simulink model "ENV"  (R2024b)
settings: Solver=FixedStepDiscrete  StartTime=0.0  StopTime=1  FixedStep=0.001  RelTol=1e-3  EnableMultiTasking=on
libraries: stm32blockslib x92, canmsglib x40, simulink x7, stm32f4xxblockslib x6
(part 1 of 5)
settings Model: DataDictionary=Master_Dictionary.sldd  STM32="{\"DigitalPortRead\":[{\"ID\":\"ENV:620\"},{\"ID\":\"ENV:1851\"},{\"ID\":\"ENV:1904\"},{\"ID\":\"ENV:2058\"}],\"SPIControllerTransfer\":[{\"ID\":\"ENV:1674\"},{\"ID\":\"ENV:1677\"},{\"ID\":\"ENV:1680\"},{\"ID\":\"ENV:1683\"},{\"ID\":\"ENV:1686\"},{\"ID\":\"ENV:1689\"},{\"ID\":\"ENV:1787\"},{\"ID\":\"ENV:1788\"},{\"ID\":\"ENV:1789\"},{\"ID\":\"ENV:1790\"},{\"ID\":\"ENV:1791\"},{\"ID\":\"ENV:1792\"},{\"ID\":\"ENV:1879\"},{\"ID\":\"ENV:1925\"},{\"ID\":\"ENV:1937\"},{\"ID\":\"ENV:1944\"},{\"ID\":\"ENV:1958\"},{\"ID\":\"ENV:1959\"},{\"ID\":\"ENV:1960\"},{\"ID\":\"ENV:1961\"},{\"ID\":\"ENV:2022\"},{\"ID\":\"ENV:2023\"},{\"ID\":\"ENV:2024\"},{\"ID\":\"ENV:2025\"},{\"ID\":\"ENV:2026\"},{\"ID\":\"ENV:2027\"},{\"ID\":\"ENV:2028\"},{\"ID\":\"ENV:2029\"},{\"ID\":\"ENV:2111\"},{\"ID\":\"ENV:2112\"},{\"ID\":\"ENV:2113\"},{\"ID\":\"ENV:2114\"},{\"ID\":\"ENV:2244\"},{\"ID\":\"ENV:2245\"},{\"ID\":\"ENV:2246\"},{\"ID\":\"ENV:2247\"},{\"ID\":\"ENV:2283\"},{\"ID\":\"ENV:2284\"},{\"ID\":\"ENV:2317\"},{\"ID\":\"ENV:2318\"},{\"ID\":\"ENV:2351\"},{\"ID\":\"ENV:2352\"},{\"ID\":\"ENV:2373\"},{\"ID\":\"ENV:2374\"},{\"ID\":\"ENV:2375\"},{\"ID\":\"ENV:2376\"},{\"ID\":\"ENV:2377\"},{\"ID\":\"ENV:2378\"},{\"ID\":\"ENV:2379\"},{\"ID\":\"ENV:2380\"},{\"ID\":\"ENV:2381\"},{\"ID\":\"ENV:2382\"},{\"ID\":\"ENV:2383\"},{\"ID\":\"ENV:2384\"},{\"ID\":\"ENV:2385\"},{\"ID\":\"ENV:2386\"},{\"ID\":\"ENV:2387\"},{\"ID\":\"ENV:2388\"},{\"ID\":\"ENV:2389\"},{\"ID\":\"ENV:2390\"},{\"ID\":\"ENV:2412\"},{\"ID\":\"ENV:2413\"},{\"ID\":\"ENV:2414\"},{\"ID\":\"ENV:2415\"},{\"ID\":\"ENV:2416\"},{\"ID\":\"ENV:2417\"},{\"ID\":\"ENV:2418\"},{\"ID\":\"ENV:2419\"},{\"ID\":\"ENV:3078\"},{\"ID\":\"ENV:3079\"},{\"ID\":\"ENV:3080\"},{\"ID\":\"ENV:3081\"},{\"ID\":\"ENV:3082\"},{\"ID\":\"ENV:3083\"},{\"ID\":\"ENV:3084\"},{\"ID\":\"ENV:3085\"},{\"ID\":\"ENV:3157\"},{\"ID\":\"ENV:3158\"},{\"ID\":\"ENV:3159\"},{\"ID\":\"ENV:3160\"},{\"ID\":\"ENV:3161\"},{\"ID\":\"ENV:3162\"},{\"ID\":\"ENV:3163\"},{\"ID\":\"ENV:3164\"},{\"ID\":\"ENV:3234\"},{\"ID\":\"ENV:3235\"},{\"ID\":\"ENV:3236\"},{\"ID\":\"ENV:3237\"},{\"ID\":\"ENV:3238\"},{\"ID\":\"ENV:3239\"},{\"ID\":\"ENV:3240\"},{\"ID\":\"ENV:3241\"}],\"DigitalPortWrite\":[{\"ID\":\"ENV:889\"},{\"ID\":\"ENV:2393\"}]}"  Creator=will  LastModifiedBy=Will
settings SolverCC: AlgebraicLoopSolver=TrustRegion
settings DataIOCC: ReturnWorkspaceOutputs=off
settings OptimizationCC: DefaultParameterBehavior=Inlined  EnhancedBackFolding=on  PassReuseOutputArgsAs=Individual arguments  ZeroExternalMemoryAtStartup=off  ZeroInternalMemoryAtStartup=off  MaxStackSize=512  OptimizeBlockOrder=speed  DifferentSizesBufferReuse=on  OptimizationCustomize=off  EfficientTunableParamExpr=on
settings DebuggingCC: ParameterTunabilityLossMsg=error  UnconnectedInputMsg=warning  UnconnectedOutputMsg=warning  UnconnectedLineMsg=warning  ArithmeticOperatorsInVariantConditions=warning
settings HardwareCC: ProdBitPerPointer=32  ProdBitPerSizeT=32  ProdBitPerPtrDiffT=32  ProdLargestAtomicInteger=Long  ProdLargestAtomicFloat=Double  ProdWordSize=32  ProdLongLongMode=on  ProdHWDeviceType=ARM Compatible->ARM Cortex-M
settings ModelReferenceCC: EnableRefExpFcnMdlSchedulingChecks=on
settings SFSimCC: MATLABDynamicMemAlloc=off  CustomCodeUndefinedFunction=UseInterfaceOnly
settings RTWCC: Description=Embedded Coder  SystemTargetFile=ert.tlc  HardwareBoard=STM32H7xx Based (Single-core)  TemplateMakefile=ert_default_tmf  CustomHeaderCode="#include \"stm32h7xx_ll_tim.h\""  CustomInitializer=LL_TIM_EnableCounter(TIM2);  Toolchain=GNU Tools for ARM Embedded Processors  GPUComputeCapability=3.5
settings CodeAppCC: ForceParamTrailComments=on  IgnoreCustomStorageClasses=off  OperatorAnnotations=on  SimulinkDataObjDesc=on  SFDataObjDesc=on  InsertBlockDesc=on
settings ERTTargetCC: TargetLangStandard=C99 (ISO)  CodeReplacementLibrary=ARM Cortex-M  ExtModeTransport=3  ExtModeStaticAlloc=on  ExtModeStaticAllocSize=2048  ExtModeMexFile=ext_xcp  ExtModeIntrfLevel=Level2 - Open

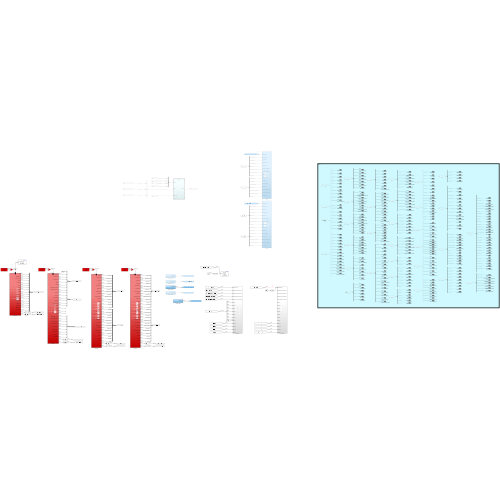
[thumbnail: Simulink's stored preview of the top-level diagram]
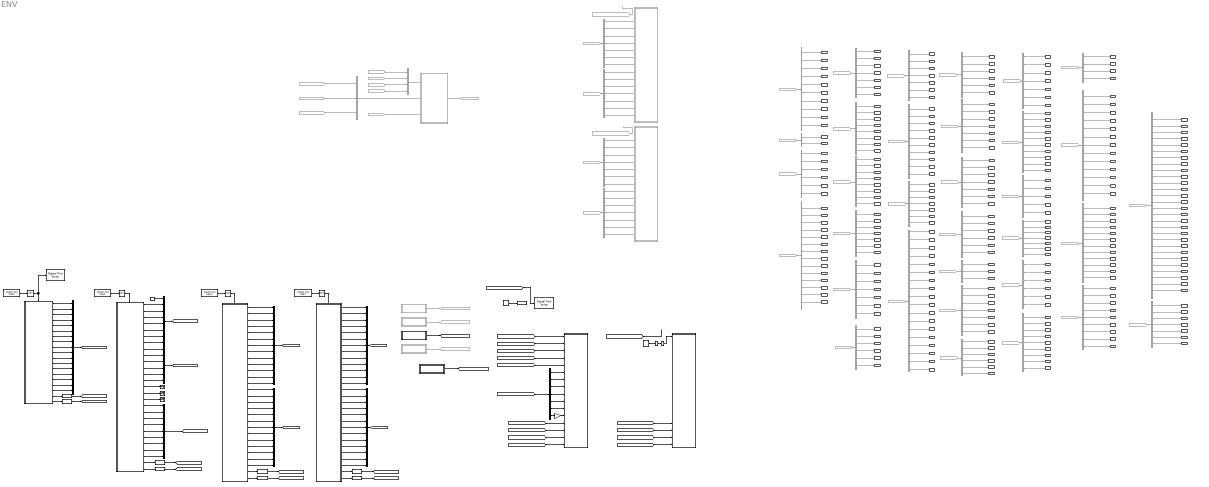
== system ENV ==
  note: CAN3
  0x1A0 : From  Commented=on  GotoTag=Global
  0x1A1 : From  Commented=on  GotoTag=Global
  0x1A2 : From  Commented=on  GotoTag=Global
  0x{202..203,205..207,210..217,220..223,250..254,300..302,603,700..703} (30 alike) : From  Commented=on  GotoTag=Global
  Bus Creator : BusCreator  Commented=on  Inputs=3  OutDataTypeStr=Bus: CAN3Bus
  Bus Creator1 : BusCreator  Inputs=8  OutDataTypeStr=Bus: DDU7
  Bus Creator14 : BusCreator  Inputs=13  OutDataTypeStr=Bus: InverterFL
  Bus Creator15 : BusCreator  Inputs=13  OutDataTypeStr=Bus: InverterFR
  Bus Creator17 : BusCreator  Inputs=13  OutDataTypeStr=Bus: InverterRL
  Bus Creator18 : BusCreator  Inputs=17  OutDataTypeStr=Bus: BMS
  Bus Creator19 : BusCreator  Inputs=13  OutDataTypeStr=Bus: InverterRR
  Bus Creator5 : BusCreator  Inputs=6  OutDataTypeStr=Bus: IMU
      settings: InheritFromInputs=off
  Bus Creator6 : BusCreator  Inputs=9  OutDataTypeStr=Bus: STW
  Bus Selector : BusSelector  Commented=on  OutputSignals=TorqueControl.MFLFinal,TorqueControl.MFRFinal,TorqueControl.MRLFinal,TorqueControl.MRRFinal,BMSSignals.IIVTS,Systems.PActual,Systems.BBrakeError,Systems.BThrottleError,Systems.BOverpower,Limitations.BDischargeAllowed
  Bus Selector1 : BusSelector  Commented=on  OutputSignals=Systems.vChassis,Systems.PEnergyMeter
  Bus Selector10 : BusSelector  Commented=on  OutputSignals=TorqueControl.MTotalRequested,TorqueControl.rSlipRatioOptimal,TorqueControl.aCamberFL,TorqueControl.aCamberFR,TorqueControl.aCamberRL,TorqueControl.aCamberRR,TorqueControl.FTotalLateralLoadTransfer
  Bus Selector11 : BusSelector  Commented=on  OutputSignals=Systems.BTVOnEM,Systems.BTVOnOW,Systems.BDrivetrainCoolingOn,Systems.BDrivetrainCoolingOnEM,Systems.BDrivetrainCoolingOnOW,Systems.BTCOn,Systems.BTCOnEM,Systems.BTCOnOW,Systems.BEMSOn,Systems.BEMSOnEM,Systems.BEMSOnOW,Systems.BSpinningModeOn,Systems.BSpinningModeOnEM,Systems.BSpinningModeOnOW,Systems.rSOE,BMSSignals.BBalancingOn,BMSSignals.BBMSP0A0C,BMSSignals.BBMSP0A0E,BMSSignals.BBMSP0A10,BMSSignals.BBMSP0A80,BMSSignals.BBMSP0AC0,BMSSignals.BBMSP0AFA,TorqueControl.NLap,Systems.NEventMode,Systems.rTorqueSplit,Systems.NThrottleMap,Systems.NThrottleMapEM,Systems.NThrottleMapOW
  Bus Selector12 : BusSelector  Commented=on  OutputSignals=Systems.aSteeringAngle,Limitations.PLowCellVoltageDischargeDerate,Limitations.PHighCellVoltageRegenDerate,TorqueControl.MDriverDischargeRequested,TorqueControl.MDriverRegenRequested,TorqueControl.PPCIntegralTermDischarge,TorqueControl.PPCIntegralTermRegen
  Bus Selector13 : BusSelector  Commented=on  OutputSignals=Stateflow.NInvState,Systems.BInverterErrorRear,Systems.BInverterErrorFront,Systems.BErrorReset,InverterSignals.InverterRLSignals.TInvRL,InverterSignals.InverterFRSignals.TMotorFR,BMSSignals.VDCAccumulator,TorqueControl.EBudget,TorqueControl.BTVOK,TorqueControl.sSector
  Bus Selector14 : BusSelector  Commented=on  OutputSignals=Systems.sChassis,Limitations.PInvTemperatureDerate,Limitations.PInvTemperatureDerateFR,Limitations.PInvTemperatureDerateFL,Limitations.PInvTemperatureDerateRR,BMSSignals.IBMSHallEffect
  Bus Selector15 : BusSelector  Commented=on  OutputSignals=TorqueControl.NABSMultiplierRR,TorqueControl.MTractionControlRRTotal,TorqueControl.MTotalFinal,TorqueControl.rSlipRatioFLActual,TorqueControl.rSlipRatioFRActual,TorqueControl.rSlipRatioRLActual,TorqueControl.FTyreVerticalFR
  Bus Selector18 : BusSelector  Commented=on  OutputSignals=Systems.PDischargeMax,Systems.PDischargeMaxEM,Systems.PDischargeMaxOW,Systems.PEngineBraking,Systems.PEngineBrakingEM,Systems.PEngineBrakingOW,Systems.rGrip,Systems.EOffset,Systems.NTCKdSelector,Systems.NPCKpSelector,Systems.MRegenMax,Systems.rTorqueSplitEM
  Bus Selector19 : BusSelector  Commented=on  OutputSignals=Systems.tThrottleError,TorqueControl.MTorqueDistributionRR,TorqueControl.NTractionControlMultiplierRL,TorqueControl.NTractionControlMultiplierRR,TorqueControl.NABSMultiplierFL,TorqueControl.NABSMultiplierFR,TorqueControl.NABSMultiplierRL,TorqueControl.FTyreVerticalFL
  Bus Selector2 : BusSelector  Commented=on  OutputSignals=WheelSpeeds.vWheelFL,WheelSpeeds.vWheelFR,InverterSignals.InverterFLSignals.nMotorFL,InverterSignals.InverterFRSignals.nMotorFR,Systems.rThrottlePedal1,Systems.BPageUp,InverterSignals.InverterRLSignals.BQuitInvOnRL,InverterSignals.InverterFLSignals.BQuitInvOnFL,InverterSignals.InverterRRSignals.BQuitInvOnRR,InverterSignals.InverterFRSignals.BQuitInvOnFR,Stateflow.BInvErrorResetRL,Stateflow.BInvErrorResetRR,Stateflow.BInvErrorResetFL,Stateflow.BInvErrorResetFR
  Bus Selector20 : BusSelector  Commented=on  OutputSignals=Stateflow.BInvDCOnRLOut,Stateflow.BInvEnableRL,Stateflow.BInvErrorResetRL,Stateflow.BInvOnRLOut,Stateflow.MTorqueLimitNegativeRL,Stateflow.MTorqueLimitPositiveRL,TorqueControl.MRLFinal
  Bus Selector21 : BusSelector  Commented=on  OutputSignals=Stateflow.BInvDCOnFLOut,Stateflow.BInvEnableFL,Stateflow.BInvErrorResetFL,Stateflow.BInvOnFLOut,Stateflow.MTorqueLimitNegativeFL,Stateflow.MTorqueLimitPositiveFL,TorqueControl.MFLFinal
  Bus Selector22 : BusSelector  Commented=on  OutputSignals=Stateflow.BInvDCOnRROut,Stateflow.BInvEnableRR,Stateflow.BInvErrorResetRR,Stateflow.BInvOnRROut,Stateflow.MTorqueLimitNegativeRR,Stateflow.MTorqueLimitPositiveRR,TorqueControl.MRRFinal
  Bus Selector23 : BusSelector  Commented=on  OutputSignals=Stateflow.BInvDCOnFROut,Stateflow.BInvEnableFR,Stateflow.BInvErrorResetFR,Stateflow.BInvOnFROut,Stateflow.MTorqueLimitNegativeFR,Stateflow.MTorqueLimitPositiveFR,TorqueControl.MFRFinal
  Bus Selector24 : BusSelector  Commented=on  OutputSignals=Systems.tBrakeError,TorqueControl.nYawRateErrorActual,TorqueControl.MTorqueDistributionRL,TorqueControl.MTractionControlRLTotal,TorqueControl.MTractionControlFRTotal,TorqueControl.MTractionControlFLTotal,TorqueControl.rSlipRatioRRActual
  Bus Selector29 : BusSelector  Commented=on  OutputSignals=Stateflow.NCarState,Systems.pBrakeF,Systems.pBrakeR,Systems.tAppsTimer,BMSSignals.VCellMax,BMSSignals.VCellMin,Limitations.PSOCDischargeDerate
  Bus Selector3 : BusSelector  Commented=on  OutputSignals=WheelSpeeds.vWheelRL,WheelSpeeds.vWheelRR,InverterSignals.InverterRLSignals.nMotorRL,InverterSignals.InverterRRSignals.nMotorRR,Systems.rThrottlePedal,Systems.BPageDown
  Bus Selector30 : BusSelector  Commented=on  OutputSignals=Limitations.rSpeedRegenDerateRL,Limitations.rSpeedRegenDerateFR,Limitations.rSpeedRegenDerateFL,Limitations.BSpeedDerateOn,Limitations.PDischargeDerate,Limitations.PRegenDerate,TorqueControl.PRegenRequested,TorqueControl.PDischargeLimit,TorqueControl.PRegenLimit,TorqueControl.PPCDischargeRequested
  Bus Selector31 : BusSelector  Commented=on  OutputSignals=Systems.BPCComplete,Systems.BBrakeLight,Stateflow.BReadyToDriveBuzzer,Systems.BAccuFanOn,Systems.BMotorRBHFanOn,Systems.BInverterFanOn,Systems.BInvLVOn
  Bus Selector33 : BusSelector  Commented=on  OutputSignals=Systems.TMotorMax,Systems.TInvMax,InverterSignals.InverterRLSignals.TMotorRL,InverterSignals.InverterRLSignals.VDCInvRL,InverterSignals.InverterRRSignals.TMotorRR,InverterSignals.InverterFLSignals.TMotorFL
  Bus Selector34 : BusSelector  Commented=on  OutputSignals=TorqueControl.ETotalRequested,TorqueControl.ESector1Remaining,TorqueControl.ESector2Remaining,TorqueControl.ESector3Remaining,TorqueControl.ESector4Remaining
  Bus Selector35 : BusSelector  Commented=on  OutputSignals=TorqueControl.ERemaining,TorqueControl.FTotalDownforce,TorqueControl.aCamberGainRollF,TorqueControl.aCamberGainRollR,TorqueControl.aCamberGainHeaveF,TorqueControl.aCamberGainHeaveR,TorqueControl.aRollAngle
  Bus Selector38 : BusSelector  Commented=on  OutputSignals=TorqueControl.NSectorGlobal,TorqueControl.NSectorLap,TorqueControl.NSector3Remaining,TorqueControl.NSector4Remaining,TorqueControl.NSector5Remaining,TorqueControl.NSector6Remaining,TorqueControl.NSector7Remaining,TorqueControl.NSector8Remaining,TorqueControl.ESector8Remaining
  Bus Selector4 : BusSelector  Commented=on  OutputSignals=Systems.tPedalOverlap,TorqueControl.PPCProportionalTermDischarge,TorqueControl.MPCDischargeRequested,TorqueControl.PPCProportionalTermRegen,TorqueControl.MPCRegenRequested,TorqueControl.MDischargeLimited,TorqueControl.NTractionControlMultiplierFL,TorqueControl.NTractionControlMultiplierFR
  Bus Selector42 : BusSelector  Commented=on  OutputSignals=Limitations.PInvTemperatureDerateRL,Limitations.PMotorTemperatureDerate,Limitations.PMotorTemperatureDerateFR,Limitations.PMotorTemperatureDerateFL,Limitations.PMotorTemperatureDerateRR,TorqueControl.aCamberGainSteerFL,TorqueControl.aCamberGainSteerFR
  Bus Selector47 : BusSelector  Commented=on  OutputSignals=Limitations.PMotorTemperatureDerateRL,Limitations.PTSTemperatureDerateFR,Limitations.PTSTemperatureDerateFL,Limitations.PTSTemperatureDerateRR,Limitations.PTSTemperatureDerateRL,Limitations.PHighCellTemperatureDerate
  Bus Selector48 : BusSelector  Commented=on  OutputSignals=TorqueControl.ESector,TorqueControl.xHeaveTravelF,TorqueControl.xHeaveTravelR
  Bus Selector49 : BusSelector  Commented=on  OutputSignals=Stateflow.NBMSState,InverterSignals.InverterRRSignals.TInvRR,InverterSignals.InverterFLSignals.TInvFL,InverterSignals.InverterFRSignals.TInvFR,BMSSignals.TCellMax,BMSSignals.TCellMin,TorqueControl.rSplitRear
  Bus Selector5 : BusSelector  Commented=on  OutputSignals=Systems.pBrakeMax,Systems.rRegenPaddle,Systems.xDamperFL,Systems.xDamperFR,Systems.xDamperRL,Systems.xDamperRR,Systems.BIMUOK,Systems.tIMUError,Systems.BDataMark
  Bus Selector53 : BusSelector  Commented=on  OutputSignals=TorqueControl.ESector9Remaining,TorqueControl.ESector10Remaining,TorqueControl.ESector11Remaining,TorqueControl.ESector12Remaining,TorqueControl.NSector1Remaining,TorqueControl.NSector2Remaining
  Bus Selector54 : BusSelector  Commented=on  OutputSignals=TorqueControl.NSector9Remaining,TorqueControl.NSector10Remaining,TorqueControl.NSector11Remaining,TorqueControl.NSector12Remaining,TorqueControl.ESector5Remaining,TorqueControl.ESector6Remaining,TorqueControl.ESector7Remaining
  Bus Selector55 : BusSelector  Commented=on  OutputSignals=Systems.rTorqueSplitOW,Systems.PRegenMax,Systems.PRegenMaxEM,Systems.PRegenMaxOW,Systems.rTVMultiplier,Systems.rTVMultiplierEM,Systems.rTVMultiplierOW,Systems.rEngineBrakingSplit,Systems.rEngineBrakingSplitEM,Systems.rEngineBrakingSplitOW,Systems.rSOC,Stateflow.BReadyToDrive,Systems.BTVOn
  Bus Selector6 : BusSelector  Commented=on  OutputSignals=TorqueControl.FTyreVerticalRL,TorqueControl.FTyreVerticalRR,TorqueControl.aSlipAngleFL,TorqueControl.aSlipAngleFR,TorqueControl.aSlipAngleRL,TorqueControl.aSlipAngleRR
  Bus Selector7 : BusSelector  Commented=on  OutputSignals=InverterSignals.InverterRLSignals.NInvDTCRL,InverterSignals.InverterRRSignals.NInvDTCRR,InverterSignals.InverterFLSignals.NInvDTCFL,InverterSignals.InverterFRSignals.NInvDTCFR
  Bus Selector8 : BusSelector  Commented=on  OutputSignals=Systems.BBrakeOn,Systems.BPedalOverlap,Systems.BAppsOK,Systems.BRegenOn,Systems.BxDamperFLOk,Systems.BxDamperFROk,Systems.BxDamperRLOk,Systems.BxDamperRROk,Systems.BIMUError,Systems.BCalibrationOn,Limitations.PSOCRegenDerate,Limitations.rSpeedRegenDerateRR,TorqueControl.PPCRegenRequested,TorqueControl.PDischargeLimited,TorqueControl.BEMSDriverSignal1,TorqueControl.BEMSDriverSignal2,TorqueControl.BEMSDriverSignal3,TorqueControl.FLongitudinalLoadTransfer
  Bus Selector9 : BusSelector  Commented=on  OutputSignals=TorqueControl.MTorqueVectoringFL,TorqueControl.MTorqueVectoringFR,TorqueControl.MTorqueVectoringRL,TorqueControl.MTorqueVectoringRR,TorqueControl.MTorqueDistributionFL,TorqueControl.MTorqueDistributionFR,TorqueControl.MRegenLimited
  CAN Tx2 : Subsystem
  CAN Tx3 : Subsystem
  CAN1 RX : Subsystem  TreatAsAtomicUnit=on
  CAN1 TX : Subsystem  Commented=on
  CAN1_2Bus : BusCreator  Commented=on  Inputs=4  OutDataTypeStr=Bus: CAN1_2Bus
  CAN2 RX : Subsystem  TreatAsAtomicUnit=on
  CAN2 TX : Subsystem  Commented=on
  CAN3 RX : Subsystem  TreatAsAtomicUnit=on
  CAN4 RX : Subsystem  TreatAsAtomicUnit=on
  Compare To Constant : simulink/Logic and Bit Operations/Compare To Constant  relop=>=  const=125  OutDataTypeStr=boolean
  Constant : Constant  OutDataTypeStr=boolean
  Constant1 : Constant  Value=69
  Counter Limited : simulink/Sources/Counter Limited  uplimit=250  tsamp=-1
  Data Type Conversion{,1..7} (8 alike) : DataTypeConversion  OutDataTypeStr=double  SaturateOnIntegerOverflow=off  RndMeth=Floor
  Demux : Demux  Outputs=7
  Digital Port Read1 : stm32f4xxblockslib/Digital Port Read  PortName=GPIOA  PinNumber=2  ReadOperation=on  IOAsArray=off  SampleTime=-1  EnableSimPort=off  hoistedMaskSrc=ECSoC/ECSimCodegen/Digital Port Read
      settings: LibrarySourceBlock=stm32f2xxblockslib/Digital Port Read
  Digital Port Read2 : stm32f4xxblockslib/Digital Port Read  PortName=GPIOC  PinNumber=4  ReadOperation=on  IOAsArray=off  SampleTime=-1  EnableSimPort=off  hoistedMaskSrc=ECSoC/ECSimCodegen/Digital Port Read
      settings: LibrarySourceBlock=stm32f2xxblockslib/Digital Port Read
  Digital Port Read3 : stm32f4xxblockslib/Digital Port Read  PortName=GPIOC  PinNumber=12  ReadOperation=on  IOAsArray=off  SampleTime=-1  EnableSimPort=off  hoistedMaskSrc=ECSoC/ECSimCodegen/Digital Port Read
      settings: LibrarySourceBlock=stm32f2xxblockslib/Digital Port Read
  Digital Port Read4 : stm32f4xxblockslib/Digital Port Read  PortName=GPIOB  PinNumber=2  ReadOperation=on  IOAsArray=off  SampleTime=-1  EnableSimPort=off  hoistedMaskSrc=ECSoC/ECSimCodegen/Digital Port Read
      settings: LibrarySourceBlock=stm32f2xxblockslib/Digital Port Read
  Digital Port Write : stm32f4xxblockslib/Digital Port Write  PortName=GPIOB  PinNumber=4  ReadOperation=off  IOAsArray=off  EnableSimPort=off  hoistedMaskSrc=ECSoC/ECSimCodegen/Digital Port Write
      settings: LibrarySourceBlock=stm32h7xxblockslib/Digital Port Write
  Digital Port Write1 : stm32f4xxblockslib/Digital Port Write  PortName=GPIOB  PinNumber=5  ReadOperation=off  IOAsArray=off  EnableSimPort=off  hoistedMaskSrc=ECSoC/ECSimCodegen/Digital Port Write
      settings: LibrarySourceBlock=stm32h7xxblockslib/Digital Port Write
  From10 : From  Commented=on  GotoTag=InverterRL
  From11 : From  Commented=on  GotoTag=DDU7
  From12 : From  Commented=on  GotoTag=STW
  From13 : From  Commented=on  GotoTag=IMU
  From18 : From  Commented=on  GotoTag=CAN1Initialized
  From19 : From  Commented=on  GotoTag=CAN2Initialized
  From6 : From  Commented=on  GotoTag=BMS
  From7 : From  Commented=on  GotoTag=InverterFL
  From8 : From  Commented=on  GotoTag=InverterFR
  From9 : From  Commented=on  GotoTag=InverterRR
  Gain : Gain  Gain=9.183
  Goto10 : Goto  Commented=on  GotoTag=CAN1Initialized
  Goto11 : Goto  Commented=on  GotoTag=CAN2Initialized
  Goto17 : Goto  Commented=on  GotoTag=Global
  Goto21 : Goto  Commented=on  GotoTag=CAN4Initialized
  INV1_Recieve_1 : From  Commented=on  GotoTag=Global
  INV2_Recieve_1 : From  Commented=on  GotoTag=Global
  INV3_Recieve_1 : From  Commented=on  GotoTag=Global
  INV4_Recieve_1 : From  Commented=on  GotoTag=Global
  Initialize CAN1 : Subsystem  Commented=on
  Initialize CAN2 : Subsystem  Commented=on
  Initialize CAN3 : Subsystem
  Initialize CAN4 : Subsystem  Commented=on
  Initialize CAN5 : Subsystem
  Model : ModelReference  Commented=on  ModelNameDialog=MASTER.slx  SimulationMode=Normal  ModelReferenceVersion=13.12
  NOT{1..4} (4 alike) : Logic  Operator=NOT  IconShape=distinctive  AllPortsSameDT=off  OutDataTypeStr=boolean
  Terminator3 : Terminator
  Terminator4 : Terminator
  Terminator5 : Terminator
  Unit Delay1 : UnitDelay  SampleTime=-1  HasFrameUpgradeWarning=on
  Unit Delay5 : UnitDelay  SampleTime=-1  HasFrameUpgradeWarning=on
  MTotalFinal : Outport  VectorParamsAs1DForOutWhenUnconnected=off
  PActual : Outport  Port=2  VectorParamsAs1DForOutWhenUnconnected=off
  rSpeedRegenDerateRR : Outport  Port=3  VectorParamsAs1DForOutWhenUnconnected=off
  PDischargeMax : Outport  Port=4  VectorParamsAs1DForOutWhenUnconnected=off
  rThrottlePedal : Outport  Port=5  VectorParamsAs1DForOutWhenUnconnected=off
  rThrottlePedal1 : Outport  Port=6  VectorParamsAs1DForOutWhenUnconnected=off
  aSteeringAngle : Outport  Port=7  VectorParamsAs1DForOutWhenUnconnected=off
  pBrakeF : Outport  Port=8  VectorParamsAs1DForOutWhenUnconnected=off
  pBrakeR : Outport  Port=9  VectorParamsAs1DForOutWhenUnconnected=off
  BBMSP0A80Out : Outport  Port=10  VectorParamsAs1DForOutWhenUnconnected=off
  BBMSP0AC0Out : Outport  Port=11  VectorParamsAs1DForOutWhenUnconnected=off
  BBMSP0AFAOut : Outport  Port=12  VectorParamsAs1DForOutWhenUnconnected=off
  BBMSP0A0COut : Outport  Port=13  VectorParamsAs1DForOutWhenUnconnected=off
  BBMSP0A0EOut : Outport  Port=14  VectorParamsAs1DForOutWhenUnconnected=off
  BBMSP0A10Out : Outport  Port=15  VectorParamsAs1DForOutWhenUnconnected=off
  BTVOK : Outport  Port=16  VectorParamsAs1DForOutWhenUnconnected=off
  NInvDTCRROut : Outport  Port=17  VectorParamsAs1DForOutWhenUnconnected=off
  NInvDTCRLOut : Outport  Port=18  VectorParamsAs1DForOutWhenUnconnected=off
  NInvDTCFROut : Outport  Port=19  VectorParamsAs1DForOutWhenUnconnected=off
  NInvDTCFLOut : Outport  Port=20  VectorParamsAs1DForOutWhenUnconnected=off
  IIVTSOut : Outport  Port=21  VectorParamsAs1DForOutWhenUnconnected=off
  MFRFinal : Outport  Port=22  VectorParamsAs1DForOutWhenUnconnected=off
  MFLFinal : Outport  Port=23  VectorParamsAs1DForOutWhenUnconnected=off
  MRLFinal : Outport  Port=24  VectorParamsAs1DForOutWhenUnconnected=off
  MRRFinal : Outport  Port=25  VectorParamsAs1DForOutWhenUnconnected=off
  rRegenPaddle : Outport  Port=26  VectorParamsAs1DForOutWhenUnconnected=off
  vChassis : Outport  Port=27  VectorParamsAs1DForOutWhenUnconnected=off
  pBrakeMax : Outport  Port=28  VectorParamsAs1DForOutWhenUnconnected=off
  vWheelRL : Outport  Port=29  VectorParamsAs1DForOutWhenUnconnected=off
  vWheelRR : Outport  Port=30  VectorParamsAs1DForOutWhenUnconnected=off
  vWheelFL : Outport  Port=31  VectorParamsAs1DForOutWhenUnconnected=off
  vWheelFR : Outport  Port=32  VectorParamsAs1DForOutWhenUnconnected=off
  BThrottleError : Outport  Port=33  VectorParamsAs1DForOutWhenUnconnected=off
  tThrottleError : Outport  Port=34  VectorParamsAs1DForOutWhenUnconnected=off
  BBrakeError : Outport  Port=35  VectorParamsAs1DForOutWhenUnconnected=off
  tBrakeError : Outport  Port=36  VectorParamsAs1DForOutWhenUnconnected=off
  BBrakeOn : Outport  Port=37  VectorParamsAs1DForOutWhenUnconnected=off
  BPedalOverlap : Outport  Port=38  VectorParamsAs1DForOutWhenUnconnected=off
  BAppsOK : Outport  Port=39  VectorParamsAs1DForOutWhenUnconnected=off
  BRegenOn : Outport  Port=40  VectorParamsAs1DForOutWhenUnconnected=off
  BTVOn : Outport  Port=41  VectorParamsAs1DForOutWhenUnconnected=off
  rSOE : Outport  Port=42  VectorParamsAs1DForOutWhenUnconnected=off
  sChassis : Outport  Port=43  VectorParamsAs1DForOutWhenUnconnected=off
  rSOC : Outport  Port=44  VectorParamsAs1DForOutWhenUnconnected=off
  rTVMultiplier : Outport  Port=45  VectorParamsAs1DForOutWhenUnconnected=off
  PEngineBraking : Outport  Port=46  VectorParamsAs1DForOutWhenUnconnected=off
  NInvState : Outport  Port=47  VectorParamsAs1DForOutWhenUnconnected=off
  rGrip : Outport  Port=48  VectorParamsAs1DForOutWhenUnconnected=off
  rSlipRatioFRActual : Outport  Port=49  VectorParamsAs1DForOutWhenUnconnected=off
  rSlipRatioRLActual : Outport  Port=50  VectorParamsAs1DForOutWhenUnconnected=off
  rSlipRatioRRActual : Outport  Port=51  VectorParamsAs1DForOutWhenUnconnected=off
  NTractionControlMultiplierRR : Outport  Port=52  VectorParamsAs1DForOutWhenUnconnected=off
  NABSMultiplierRR : Outport  Port=53  VectorParamsAs1DForOutWhenUnconnected=off
  NTractionControlMultiplierRL : Outport  Port=54  VectorParamsAs1DForOutWhenUnconnected=off
  NABSMultiplierRL : Outport  Port=55  VectorParamsAs1DForOutWhenUnconnected=off
  NThrottleMap : Outport  Port=56  VectorParamsAs1DForOutWhenUnconnected=off
  BReadyToDrive : Outport  Port=57  VectorParamsAs1DForOutWhenUnconnected=off
  NABSMultiplierFL : Outport  Port=58  VectorParamsAs1DForOutWhenUnconnected=off
  NABSMultiplierFR : Outport  Port=59  VectorParamsAs1DForOutWhenUnconnected=off
  BBalancingOnOut : Outport  Port=60  VectorParamsAs1DForOutWhenUnconnected=off
  MTorqueVectoringFL : Outport  Port=61  VectorParamsAs1DForOutWhenUnconnected=off
  MTorqueVectoringFR : Outport  Port=62  VectorParamsAs1DForOutWhenUnconnected=off
  MTorqueVectoringRL : Outport  Port=63  VectorParamsAs1DForOutWhenUnconnected=off
  MTorqueVectoringRR : Outport  Port=64  VectorParamsAs1DForOutWhenUnconnected=off
  NTractionControlMultiplierFL : Outport  Port=65  VectorParamsAs1DForOutWhenUnconnected=off
  NTractionControlMultiplierFR : Outport  Port=66  VectorParamsAs1DForOutWhenUnconnected=off
  MDischargeLimited : Outport  Port=67  VectorParamsAs1DForOutWhenUnconnected=off
  MDriverRegenRequested : Outport  Port=68  VectorParamsAs1DForOutWhenUnconnected=off
  rSlipRatioOptimal : Outport  Port=69  VectorParamsAs1DForOutWhenUnconnected=off
  NCarState : Outport  Port=70  VectorParamsAs1DForOutWhenUnconnected=off
  MTorqueDistributionFL : Outport  Port=71  VectorParamsAs1DForOutWhenUnconnected=off
  MTorqueDistributionFR : Outport  Port=72  VectorParamsAs1DForOutWhenUnconnected=off
  MTorqueDistributionRL : Outport  Port=73  VectorParamsAs1DForOutWhenUnconnected=off
  MTorqueDistributionRR : Outport  Port=74  VectorParamsAs1DForOutWhenUnconnected=off
  nMotorRLOut : Outport  Port=75  VectorParamsAs1DForOutWhenUnconnected=off
  nMotorFLOut : Outport  Port=76  VectorParamsAs1DForOutWhenUnconnected=off
  nMotorRROut : Outport  Port=77  VectorParamsAs1DForOutWhenUnconnected=off
  nMotorFROut : Outport  Port=78  VectorParamsAs1DForOutWhenUnconnected=off
  BDischargeAllowed : Outport  Port=79  VectorParamsAs1DForOutWhenUnconnected=off
  TMotorRLOut : Outport  Port=80  VectorParamsAs1DForOutWhenUnconnected=off
  TInvRLOut : Outport  Port=81  VectorParamsAs1DForOutWhenUnconnected=off
  TMotorFLOut : Outport  Port=82  VectorParamsAs1DForOutWhenUnconnected=off
  TInvFLOut : Outport  Port=83  VectorParamsAs1DForOutWhenUnconnected=off
  TMotorRROut : Outport  Port=84  VectorParamsAs1DForOutWhenUnconnected=off
  TInvRROut : Outport  Port=85  VectorParamsAs1DForOutWhenUnconnected=off
  TMotorFROut : Outport  Port=86  VectorParamsAs1DForOutWhenUnconnected=off
  TInvFROut : Outport  Port=87  VectorParamsAs1DForOutWhenUnconnected=off
  TInvMax : Outport  Port=88  VectorParamsAs1DForOutWhenUnconnected=off
  TMotorMax : Outport  Port=89  VectorParamsAs1DForOutWhenUnconnected=off
  TCellMaxOut : Outport  Port=90  VectorParamsAs1DForOutWhenUnconnected=off
  IBMSHallEffectOut : Outport  Port=91  VectorParamsAs1DForOutWhenUnconnected=off
  VDCInvRLOut : Outport  Port=92  VectorParamsAs1DForOutWhenUnconnected=off
  BEMSOn : Outport  Port=93  VectorParamsAs1DForOutWhenUnconnected=off
  BTCOn : Outport  Port=94  VectorParamsAs1DForOutWhenUnconnected=off
  VCellMinOut : Outport  Port=95  VectorParamsAs1DForOutWhenUnconnected=off
  VCellMaxOut : Outport  Port=96  VectorParamsAs1DForOutWhenUnconnected=off
  TCellMinOut : Outport  Port=97  VectorParamsAs1DForOutWhenUnconnected=off
  nYawRateErrorActual : Outport  Port=98  VectorParamsAs1DForOutWhenUnconnected=off
  tPedalOverlap : Outport  Port=99  VectorParamsAs1DForOutWhenUnconnected=off
  tAppsTimer : Outport  Port=100  VectorParamsAs1DForOutWhenUnconnected=off
  rSplitRear : Outport  Port=101  VectorParamsAs1DForOutWhenUnconnected=off
  PRegenLimit : Outport  Port=102  VectorParamsAs1DForOutWhenUnconnected=off
  PRegenRequested : Outport  Port=103  VectorParamsAs1DForOutWhenUnconnected=off
  BIMUOk : Outport  Port=104  VectorParamsAs1DForOutWhenUnconnected=off
  EOffset : Outport  Port=105  VectorParamsAs1DForOutWhenUnconnected=off
  PEnergyMeter : Outport  Port=106  VectorParamsAs1DForOutWhenUnconnected=off
  NBMSState : Outport  Port=107  VectorParamsAs1DForOutWhenUnconnected=off
  BOverpower : Outport  Port=108  VectorParamsAs1DForOutWhenUnconnected=off
  BPCComplete : Outport  Port=109  VectorParamsAs1DForOutWhenUnconnected=off
  BEMSDriverSignal1 : Outport  Port=110  VectorParamsAs1DForOutWhenUnconnected=off
  BEMSDriverSignal2 : Outport  Port=111  VectorParamsAs1DForOutWhenUnconnected=off
  BEMSDriverSignal3 : Outport  Port=112  VectorParamsAs1DForOutWhenUnconnected=off
  BPageUp : Outport  Port=113  VectorParamsAs1DForOutWhenUnconnected=off
  BPageDown : Outport  Port=114  VectorParamsAs1DForOutWhenUnconnected=off
  MRegenMax : Outport  Port=115  VectorParamsAs1DForOutWhenUnconnected=off
  NSectorLap : Outport  Port=116  VectorParamsAs1DForOutWhenUnconnected=off
  MPCRegenRequested : Outport  Port=117  VectorParamsAs1DForOutWhenUnconnected=off
  MPCDischargeRequested : Outport  Port=118  VectorParamsAs1DForOutWhenUnconnected=off
  PPCIntegralTermDischarge : Outport  Port=119  VectorParamsAs1DForOutWhenUnconnected=off
  PPCIntegralTermRegen : Outport  Port=120  VectorParamsAs1DForOutWhenUnconnected=off
  NSectorGlobal : Outport  Port=121  VectorParamsAs1DForOutWhenUnconnected=off
  PPCProportionalTermDischarge : Outport  Port=122  VectorParamsAs1DForOutWhenUnconnected=off
  PPCProportionalTermRegen : Outport  Port=123  VectorParamsAs1DForOutWhenUnconnected=off
  BDataMark : Outport  Port=124  VectorParamsAs1DForOutWhenUnconnected=off
  xDamperFL : Outport  Port=125  VectorParamsAs1DForOutWhenUnconnected=off
  xDamperFR : Outport  Port=126  VectorParamsAs1DForOutWhenUnconnected=off
  xDamperRR : Outport  Port=127  VectorParamsAs1DForOutWhenUnconnected=off
  xDamperRL : Outport  Port=128  VectorParamsAs1DForOutWhenUnconnected=off
  BErrorReset : Outport  Port=129  VectorParamsAs1DForOutWhenUnconnected=off
  BDrivetrainCoolingOn : Outport  Port=130  VectorParamsAs1DForOutWhenUnconnected=off
  PPCRegenRequested : Outport  Port=131  VectorParamsAs1DForOutWhenUnconnected=off
  PDischargeLimit : Outport  Port=132  VectorParamsAs1DForOutWhenUnconnected=off
  PRegenDerate : Outport  Port=133  VectorParamsAs1DForOutWhenUnconnected=off
  PHighCellVoltageRegenDerate : Outport  Port=134  VectorParamsAs1DForOutWhenUnconnected=off
  PHighCellTemperatureDerate : Outport  Port=135  VectorParamsAs1DForOutWhenUnconnected=off
  PDischargeDerate : Outport  Port=136  VectorParamsAs1DForOutWhenUnconnected=off
  PMotorTemperatureDerate : Outport  Port=137  VectorParamsAs1DForOutWhenUnconnected=off
  PMotorTemperatureDerateFL : Outport  Port=138  VectorParamsAs1DForOutWhenUnconnected=off
  PMotorTemperatureDerateFR : Outport  Port=139  VectorParamsAs1DForOutWhenUnconnected=off
  PMotorTemperatureDerateRL : Outport  Port=140  VectorParamsAs1DForOutWhenUnconnected=off
  PMotorTemperatureDerateRR : Outport  Port=141  VectorParamsAs1DForOutWhenUnconnected=off
  PLowCellVoltageDischargeDerate : Outport  Port=142  VectorParamsAs1DForOutWhenUnconnected=off
  PInvTemperatureDerate : Outport  Port=143  VectorParamsAs1DForOutWhenUnconnected=off
  PInvTemperatureDerateFL : Outport  Port=144  VectorParamsAs1DForOutWhenUnconnected=off
  PInvTemperatureDerateFR : Outport  Port=145  VectorParamsAs1DForOutWhenUnconnected=off
  PInvTemperatureDerateRR : Outport  Port=146  VectorParamsAs1DForOutWhenUnconnected=off
  PInvTemperatureDerateRL : Outport  Port=147  VectorParamsAs1DForOutWhenUnconnected=off
  aCamberGainSteerFL : Outport  Port=148  VectorParamsAs1DForOutWhenUnconnected=off
  aCamberGainSteerFR : Outport  Port=149  VectorParamsAs1DForOutWhenUnconnected=off
  PPCDischargeRequested : Outport  Port=150  VectorParamsAs1DForOutWhenUnconnected=off
  rSlipRatioFLActual : Outport  Port=151  VectorParamsAs1DForOutWhenUnconnected=off
  FLongitudinalLoadTransfer : Outport  Port=152  VectorParamsAs1DForOutWhenUnconnected=off
  FTyreVerticalFL : Outport  Port=153  VectorParamsAs1DForOutWhenUnconnected=off
  FTyreVerticalFR : Outport  Port=154  VectorParamsAs1DForOutWhenUnconnected=off
  FTyreVerticalRL : Outport  Port=155  VectorParamsAs1DForOutWhenUnconnected=off
  FTyreVerticalRR : Outport  Port=156  VectorParamsAs1DForOutWhenUnconnected=off
  BCalibrationOn : Outport  Port=157  VectorParamsAs1DForOutWhenUnconnected=off
  FTotalDownforce : Outport  Port=158  VectorParamsAs1DForOutWhenUnconnected=off
  aSlipAngleFL : Outport  Port=159  VectorParamsAs1DForOutWhenUnconnected=off
  aSlipAngleFR : Outport  Port=160  VectorParamsAs1DForOutWhenUnconnected=off
  aCamberFL : Outport  Port=161  VectorParamsAs1DForOutWhenUnconnected=off
  aCamberFR : Outport  Port=162  VectorParamsAs1DForOutWhenUnconnected=off
  aCamberRL : Outport  Port=163  VectorParamsAs1DForOutWhenUnconnected=off
  aCamberRR : Outport  Port=164  VectorParamsAs1DForOutWhenUnconnected=off
  aRollAngle : Outport  Port=165  VectorParamsAs1DForOutWhenUnconnected=off
  xHeaveTravelR : Outport  Port=166  VectorParamsAs1DForOutWhenUnconnected=off
  xHeaveTravelF : Outport  Port=167  VectorParamsAs1DForOutWhenUnconnected=off
  rSpeedRegenDerateFR : Outport  Port=168  VectorParamsAs1DForOutWhenUnconnected=off
  rSpeedRegenDerateRL : Outport  Port=169  VectorParamsAs1DForOutWhenUnconnected=off
  rSpeedRegenDerateFL : Outport  Port=170  VectorParamsAs1DForOutWhenUnconnected=off
  PTSTemperatureDerateFL : Outport  Port=171  VectorParamsAs1DForOutWhenUnconnected=off
  PTSTemperatureDerateFR : Outport  Port=172  VectorParamsAs1DForOutWhenUnconnected=off
  PTSTemperatureDerateRL : Outport  Port=173  VectorParamsAs1DForOutWhenUnconnected=off
  PTSTemperatureDerateRR : Outport  Port=174  VectorParamsAs1DForOutWhenUnconnected=off
  PSOCDischargeDerate : Outport  Port=175  VectorParamsAs1DForOutWhenUnconnected=off
  PSOCRegenDerate : Outport  Port=176  VectorParamsAs1DForOutWhenUnconnected=off
  aSlipAngleRL : Outport  Port=177  VectorParamsAs1DForOutWhenUnconnected=off
  aSlipAngleRR : Outport  Port=178  VectorParamsAs1DForOutWhenUnconnected=off
  BSpeedDerateOn : Outport  Port=179  VectorParamsAs1DForOutWhenUnconnected=off
  VDCAccumulatorOut : Outport  Port=180  VectorParamsAs1DForOutWhenUnconnected=off
  MTractionControlRRTotal : Outport  Port=181  VectorParamsAs1DForOutWhenUnconnected=off
  MTractionControlRLTotal : Outport  Port=182  VectorParamsAs1DForOutWhenUnconnected=off
  MTractionControlFRTotal : Outport  Port=183  VectorParamsAs1DForOutWhenUnconnected=off
  MTractionControlFLTotal : Outport  Port=184  VectorParamsAs1DForOutWhenUnconnected=off
  BSpinningModeOn : Outport  Port=185  VectorParamsAs1DForOutWhenUnconnected=off
  PRegenMax : Outport  Port=186  VectorParamsAs1DForOutWhenUnconnected=off
  rEngineBrakingSplit : Outport  Port=187  VectorParamsAs1DForOutWhenUnconnected=off
  NLap : Outport  Port=188  VectorParamsAs1DForOutWhenUnconnected=off
  sSector : Outport  Port=189  VectorParamsAs1DForOutWhenUnconnected=off
  EBudget : Outport  Port=190  VectorParamsAs1DForOutWhenUnconnected=off
  ERemaining : Outport  Port=191  VectorParamsAs1DForOutWhenUnconnected=off
  ESector : Outport  Port=192  VectorParamsAs1DForOutWhenUnconnected=off
  FTotalLateralLoadTransfer : Outport  Port=193  VectorParamsAs1DForOutWhenUnconnected=off
  BAccuFanOn : Outport  Port=194  VectorParamsAs1DForOutWhenUnconnected=off
  BMotorRBHFanOn : Outport  Port=195  VectorParamsAs1DForOutWhenUnconnected=off
  BInverterFanOn : Outport  Port=196  VectorParamsAs1DForOutWhenUnconnected=off
  BReadyToDriveBuzzer : Outport  Port=197  VectorParamsAs1DForOutWhenUnconnected=off
  BBrakeLight : Outport  Port=198  VectorParamsAs1DForOutWhenUnconnected=off
  BInvLVOn : Outport  Port=199  VectorParamsAs1DForOutWhenUnconnected=off
  tIMUError : Outport  Port=200  VectorParamsAs1DForOutWhenUnconnected=off
  MDriverDischargeRequested : Outport  Port=201  VectorParamsAs1DForOutWhenUnconnected=off
  MRegenLimited : Outport  Port=202  VectorParamsAs1DForOutWhenUnconnected=off
  MTotalRequested : Outport  Port=203  VectorParamsAs1DForOutWhenUnconnected=off
  BxDamperFLOk : Outport  Port=204  VectorParamsAs1DForOutWhenUnconnected=off
  BxDamperFROk : Outport  Port=205  VectorParamsAs1DForOutWhenUnconnected=off
  BxDamperRLOk : Outport  Port=206  VectorParamsAs1DForOutWhenUnconnected=off
  BxDamperRROk : Outport  Port=207  VectorParamsAs1DForOutWhenUnconnected=off
  BIMUError : Outport  Port=208  VectorParamsAs1DForOutWhenUnconnected=off
  PDischargeLimited : Outport  Port=209  VectorParamsAs1DForOutWhenUnconnected=off
  aCamberGainRollF : Outport  Port=210  VectorParamsAs1DForOutWhenUnconnected=off
  aCamberGainRollR : Outport  Port=211  VectorParamsAs1DForOutWhenUnconnected=off
  aCamberGainHeaveF : Outport  Port=212  VectorParamsAs1DForOutWhenUnconnected=off
  aCamberGainHeaveR : Outport  Port=213  VectorParamsAs1DForOutWhenUnconnected=off
  BInverterErrorRear : Outport  Port=214  VectorParamsAs1DForOutWhenUnconnected=off
  BInverterErrorFront : Outport  Port=215  VectorParamsAs1DForOutWhenUnconnected=off
  ETotalRequested : Outport  Port=216  VectorParamsAs1DForOutWhenUnconnected=off
  ESector1Remaining : Outport  Port=217  VectorParamsAs1DForOutWhenUnconnected=off
  ESector2Remaining : Outport  Port=218  VectorParamsAs1DForOutWhenUnconnected=off
  ESector3Remaining : Outport  Port=219  VectorParamsAs1DForOutWhenUnconnected=off
  ESector4Remaining : Outport  Port=220  VectorParamsAs1DForOutWhenUnconnected=off
  NSector9Remaining : Outport  Port=221  VectorParamsAs1DForOutWhenUnconnected=off
  NSector10Remaining : Outport  Port=222  VectorParamsAs1DForOutWhenUnconnected=off
  NSector11Remaining : Outport  Port=223  VectorParamsAs1DForOutWhenUnconnected=off
  NSector12Remaining : Outport  Port=224  VectorParamsAs1DForOutWhenUnconnected=off
  ESector5Remaining : Outport  Port=225  VectorParamsAs1DForOutWhenUnconnected=off
  ESector6Remaining : Outport  Port=226  VectorParamsAs1DForOutWhenUnconnected=off
  ESector7Remaining : Outport  Port=227  VectorParamsAs1DForOutWhenUnconnected=off
  ESector9Remaining : Outport  Port=228  VectorParamsAs1DForOutWhenUnconnected=off
  ESector10Remaining : Outport  Port=229  VectorParamsAs1DForOutWhenUnconnected=off
  ESector11Remaining : Outport  Port=230  VectorParamsAs1DForOutWhenUnconnected=off
  ESector12Remaining : Outport  Port=231  VectorParamsAs1DForOutWhenUnconnected=off
  NSector1Remaining : Outport  Port=232  VectorParamsAs1DForOutWhenUnconnected=off
  NSector2Remaining : Outport  Port=233  VectorParamsAs1DForOutWhenUnconnected=off
  NSector3Remaining : Outport  Port=234  VectorParamsAs1DForOutWhenUnconnected=off
  NSector4Remaining : Outport  Port=235  VectorParamsAs1DForOutWhenUnconnected=off
  NSector5Remaining : Outport  Port=236  VectorParamsAs1DForOutWhenUnconnected=off
  NSector6Remaining : Outport  Port=237  VectorParamsAs1DForOutWhenUnconnected=off
  NSector7Remaining : Outport  Port=238  VectorParamsAs1DForOutWhenUnconnected=off
  NSector8Remaining : Outport  Port=239  VectorParamsAs1DForOutWhenUnconnected=off
  ESector8Remaining : Outport  Port=240  VectorParamsAs1DForOutWhenUnconnected=off
  NThrottleMapEM : Outport  Port=241  VectorParamsAs1DForOutWhenUnconnected=off
  NThrottleMapOW : Outport  Port=242  VectorParamsAs1DForOutWhenUnconnected=off
  rTorqueSplit : Outport  Port=243  VectorParamsAs1DForOutWhenUnconnected=off
  rTorqueSplitOW : Outport  Port=244  VectorParamsAs1DForOutWhenUnconnected=off
  PRegenMaxEM : Outport  Port=245  VectorParamsAs1DForOutWhenUnconnected=off
  PRegenMaxOW : Outport  Port=246  VectorParamsAs1DForOutWhenUnconnected=off
  rTVMultiplierEM : Outport  Port=247  VectorParamsAs1DForOutWhenUnconnected=off
  rTVMultiplierOW : Outport  Port=248  VectorParamsAs1DForOutWhenUnconnected=off
  rEngineBrakingSplitEM : Outport  Port=249  VectorParamsAs1DForOutWhenUnconnected=off
  rEngineBrakingSplitOW : Outport  Port=250  VectorParamsAs1DForOutWhenUnconnected=off
  PDischargeMaxEM : Outport  Port=251  VectorParamsAs1DForOutWhenUnconnected=off
  PDischargeMaxOW : Outport  Port=252  VectorParamsAs1DForOutWhenUnconnected=off
  PEngineBrakingEM : Outport  Port=253  VectorParamsAs1DForOutWhenUnconnected=off
  PEngineBrakingOW : Outport  Port=254  VectorParamsAs1DForOutWhenUnconnected=off
  NTCKdSelector : Outport  Port=255  VectorParamsAs1DForOutWhenUnconnected=off
  NPCKpSelector : Outport  Port=256  VectorParamsAs1DForOutWhenUnconnected=off
  rTorqueSplitEM : Outport  Port=257  VectorParamsAs1DForOutWhenUnconnected=off
  BTVOnEM : Outport  Port=258  VectorParamsAs1DForOutWhenUnconnected=off
  BTVOnOW : Outport  Port=259  VectorParamsAs1DForOutWhenUnconnected=off
  BDrivetrainCoolingOnEM : Outport  Port=260  VectorParamsAs1DForOutWhenUnconnected=off
  BDrivetrainCoolingOnOW : Outport  Port=261  VectorParamsAs1DForOutWhenUnconnected=off
  BTCOnEM : Outport  Port=262  VectorParamsAs1DForOutWhenUnconnected=off
  BTCOnOW : Outport  Port=263  VectorParamsAs1DForOutWhenUnconnected=off
  BEMSOnEM : Outport  Port=264  VectorParamsAs1DForOutWhenUnconnected=off
  BEMSOnOW : Outport  Port=265  VectorParamsAs1DForOutWhenUnconnected=off
  BSpinningModeOnEM : Outport  Port=266  VectorParamsAs1DForOutWhenUnconnected=off
  BSpinningModeOnOW : Outport  Port=267  VectorParamsAs1DForOutWhenUnconnected=off
  NEventMode : Outport  Port=268  VectorParamsAs1DForOutWhenUnconnected=off
  BInvErrorResetRLCAN3 : Outport  Port=269  VectorParamsAs1DForOutWhenUnconnected=off
  BInvErrorResetFLCAN3 : Outport  Port=270  VectorParamsAs1DForOutWhenUnconnected=off
  BInvErrorResetFRCAN3 : Outport  Port=271  VectorParamsAs1DForOutWhenUnconnected=off
  BInvErrorResetRRCAN3 : Outport  Port=272  VectorParamsAs1DForOutWhenUnconnected=off
  BQuitInvOnFLCAN3 : Outport  Port=273  VectorParamsAs1DForOutWhenUnconnected=off
  BQuitInvOnFRCAN3 : Outport  Port=274  VectorParamsAs1DForOutWhenUnconnected=off
  BQuitInvOnRRCAN3 : Outport  Port=275  VectorParamsAs1DForOutWhenUnconnected=off
  BQuitInvOnRLCAN3 : Outport  Port=276  VectorParamsAs1DForOutWhenUnconnected=off
  wires:
  Digital Port Read1/1 -> NOT4/1
  Initialize CAN3/1(MCPInitialized) -> [CAN3Initialized]
  Counter Limited/1 -> Compare To Constant/1
  [CAN4Initialized] -> Digital Port Write/1
  Bus Selector4/5 -> MPCRegenRequested/1  "<MPCRegenRequested>"
  Bus Selector54/1 -> NSector9Remaining/1  "<NSector9Remaining>"
  INV1_Recieve_1/1 -> Bus Selector20/1
  Bus Selector11/12 -> BSpinningModeOn/1  "<BSpinningModeOn>"
  0x302/1 -> Bus Selector13/1
  Bus Selector55/11 -> rSOC/1  "<rSOC>"
  Bus Selector2/4 -> nMotorFROut/1  "<nMotorFR>"
  Bus Selector4/1 -> tPedalOverlap/1  "<tPedalOverlap>"
  Bus Selector35/5 -> aCamberGainHeaveF/1  "<aCamberGainHeaveF>"
  Bus Selector29/1 -> NCarState/1  "<NCarState>"
  Bus Selector33/3 -> TMotorRLOut/1  "<TMotorRL>"
  Bus Selector21/4 -> CAN2 TX/5(BInvOnFLOut)  "<BInvOnFLOut>"
  Bus Selector12/3 -> PHighCellVoltageRegenDerate/1  "<PHighCellVoltageRegenDerate>"
  Bus Selector5/6 -> xDamperRR/1  "<xDamperRR>"
  From9/1 -> CAN1_2Bus/4  "InverterRR"
  Bus Selector38/6 -> NSector6Remaining/1  "<NSector6Remaining>"
  Bus Selector38/5 -> NSector5Remaining/1  "<NSector5Remaining>"
  Bus Selector42/6 -> aCamberGainSteerFL/1  "<aCamberGainSteerFL>"
  Bus Selector2/13 -> BInvErrorResetFLCAN3/1  "<BInvErrorResetFL>"
  Bus Selector15/1 -> NABSMultiplierRR/1  "<NABSMultiplierRR>"
  Bus Selector29/6 -> VCellMinOut/1  "<VCellMin>"
  Bus Selector5/5 -> xDamperRL/1  "<xDamperRL>"
  From6/1 -> Model/3
  0x217/1 -> Bus Selector6/1
  Bus Selector31/3 -> BReadyToDriveBuzzer/1  "<BReadyToDriveBuzzer>"
  Bus Selector22/4 -> CAN1 TX/12(BInvOnRROut)  "<BInvOnRROut>"
  Bus Selector20/4 -> CAN1 TX/5(BInvOnRLOut)  "<BInvOnRLOut>"
  Bus Selector8/17 -> BEMSDriverSignal3/1  "<BEMSDriverSignal3>"
  Bus Selector30/4 -> BSpeedDerateOn/1  "<BSpeedDerateOn>"
  Bus Selector35/1 -> ERemaining/1  "<ERemaining>"
  Bus Selector14/5 -> PInvTemperatureDerateRR/1  "<PInvTemperatureDerateRR>"
  Bus Selector/3 -> MRLFinal/1  "<MRLFinal>"
  Bus Selector29/4 -> tAppsTimer/1  "<tAppsTimer>"
  Bus Selector29/3 -> pBrakeR/1  "<pBrakeR>"
  Bus Selector11/22 -> BBMSP0AFAOut/1  "<BBMSP0AFA>"
  Bus Selector5/7 -> BIMUOk/1  "<BIMUOK>"
  Bus Selector7/2 -> NInvDTCRROut/1  "<NInvDTCRR>"
  Bus Selector11/5 -> BDrivetrainCoolingOnOW/1  "<BDrivetrainCoolingOnOW>"
  Bus Selector19/7 -> NABSMultiplierRL/1  "<NABSMultiplierRL>"
  Bus Selector33/4 -> VDCInvRLOut/1  "<VDCInvRL>"
  Bus Selector19/5 -> NABSMultiplierFL/1  "<NABSMultiplierFL>"
  Bus Selector9/7 -> MRegenLimited/1  "<MRegenLimited>"
  Bus Selector55/6 -> rTVMultiplierEM/1  "<rTVMultiplierEM>"
  Bus Selector53/5 -> NSector1Remaining/1  "<NSector1Remaining>"
  Bus Selector5/1 -> pBrakeMax/1  "<pBrakeMax>"
  Bus Selector34/5 -> ESector4Remaining/1  "<ESector4Remaining>"
  Bus Selector10/1 -> MTotalRequested/1  "<MTotalRequested>"
  CAN1_2Bus/1 -> Model/1
  Bus Selector33/1 -> TMotorMax/1  "<TMotorMax>"
  Bus Selector29/7 -> PSOCDischargeDerate/1  "<PSOCDischargeDerate>"
  0x213/1 -> Bus Selector4/1
  Bus Selector18/2 -> PDischargeMaxEM/1  "<PDischargeMaxEM>"
  Bus Selector48/2 -> xHeaveTravelF/1  "<xHeaveTravelF>"
  Bus Selector55/8 -> rEngineBrakingSplit/1  "<rEngineBrakingSplit>"
  Bus Selector4/4 -> PPCProportionalTermRegen/1  "<PPCProportionalTermRegen>"
  Bus Selector8/6 -> BxDamperFROk/1  "<BxDamperFROk>"
  Bus Selector30/10 -> PPCDischargeRequested/1  "<PPCDischargeRequested>"
  Bus Selector35/6 -> aCamberGainHeaveR/1  "<aCamberGainHeaveR>"
  Bus Selector15/3 -> MTotalFinal/1  "<MTotalFinal>"
  Bus Selector38/1 -> NSectorGlobal/1  "<NSectorGlobal>"
  0x220/1 -> Bus Selector29/1
  Bus Selector55/12 -> BReadyToDrive/1  "<BReadyToDrive>"
  Bus Selector13/3 -> BInverterErrorFront/1  "<BInverterErrorFront>"
  Bus Selector14/2 -> PInvTemperatureDerate/1  "<PInvTemperatureDerate>"
  0x300/1 -> Bus Selector33/1
  Bus Selector3/3 -> nMotorRLOut/1  "<nMotorRL>"
  Bus Selector8/18 -> FLongitudinalLoadTransfer/1  "<FLongitudinalLoadTransfer>"
  Bus Selector55/7 -> rTVMultiplierOW/1  "<rTVMultiplierOW>"
  Bus Selector38/3 -> NSector3Remaining/1  "<NSector3Remaining>"
  Bus Selector18/9 -> NTCKdSelector/1  "<NTCKdSelector>"
  Bus Selector8/8 -> BxDamperRROk/1  "<BxDamperRROk>"
  Bus Selector15/4 -> rSlipRatioFLActual/1  "<rSlipRatioFLActual>"
  INV3_Recieve_1/1 -> Bus Selector22/1
  Bus Selector4/6 -> MDischargeLimited/1  "<MDischargeLimited>"
  Bus Selector3/2 -> vWheelRR/1  "<vWheelRR>"
  Bus Selector30/9 -> PRegenLimit/1  "<PRegenLimit>"
  Bus Selector2/6 -> BPageUp/1  "<BPageUp>"
  Bus Selector1/1 -> vChassis/1  "<vChassis>"
  Bus Selector5/2 -> rRegenPaddle/1  "<rRegenPaddle>"
  Bus Selector24/6 -> MTractionControlFLTotal/1  "<MTractionControlFLTotal>"
  Bus Selector/7 -> BBrakeError/1  "<BBrakeError>"
  Bus Selector4/7 -> NTractionControlMultiplierFL/1  "<NTractionControlMultiplierFL>"
  Bus Selector11/26 -> NThrottleMap/1  "<NThrottleMap>"
  Bus Selector8/10 -> BCalibrationOn/1  "<BCalibrationOn>"
  Bus Selector13/8 -> EBudget/1  "<EBudget>"
  Bus Selector47/6 -> PHighCellTemperatureDerate/1  "<PHighCellTemperatureDerate>"
  Bus Selector24/4 -> MTractionControlRLTotal/1  "<MTractionControlRLTotal>"
  Bus Selector6/1 -> FTyreVerticalRL/1  "<FTyreVerticalRL>"
  Bus Selector29/2 -> pBrakeF/1  "<pBrakeF>"
  Bus Selector47/2 -> PTSTemperatureDerateFR/1  "<PTSTemperatureDerateFR>"
  0x1A1/1 -> Bus Selector55/1
  Bus Selector55/4 -> PRegenMaxOW/1  "<PRegenMaxOW>"
  Bus Selector11/20 -> BBMSP0A80Out/1  "<BBMSP0A80>"
  0x206/1 -> Bus Selector3/1
  Bus Selector3/4 -> nMotorRROut/1  "<nMotorRR>"
  Bus Selector18/7 -> rGrip/1  "<rGrip>"
  Bus Selector35/2 -> FTotalDownforce/1  "<FTotalDownforce>"
  Bus Selector13/6 -> TMotorFROut/1  "<TMotorFR>"
  Bus Selector24/3 -> MTorqueDistributionRL/1  "<MTorqueDistributionRL>"
  Bus Selector20/1 -> CAN1 TX/2(BInvDCOnRLOut)  "<BInvDCOnRLOut>"
  0x253/1 -> Bus Selector47/1
  0x254/1 -> Bus Selector48/1
  0x214/1 -> Bus Selector19/1
  Bus Selector2/3 -> nMotorFLOut/1  "<nMotorFL>"
  Bus Selector12/4 -> MDriverDischargeRequested/1  "<MDriverDischargeRequested>"
  Bus Selector49/5 -> TCellMaxOut/1  "<TCellMax>"
  Bus Selector54/3 -> NSector11Remaining/1  "<NSector11Remaining>"
  Bus Selector54/2 -> NSector10Remaining/1  "<NSector10Remaining>"
  Bus Selector8/12 -> rSpeedRegenDerateRR/1  "<rSpeedRegenDerateRR>"
  Bus Selector20/3 -> CAN1 TX/4(BInvErrorResetRL)  "<BInvErrorResetRL>"
  0x1A0/1 -> Bus Selector11/1
  Bus Selector11/9 -> BEMSOn/1  "<BEMSOn>"
  Bus Selector53/3 -> ESector11Remaining/1  "<ESector11Remaining>"
  Bus Selector53/2 -> ESector10Remaining/1  "<ESector10Remaining>"
  Bus Selector54/4 -> NSector12Remaining/1  "<NSector12Remaining>"
  Bus Selector49/2 -> TInvRROut/1  "<TInvRR>"
  Bus Selector24/2 -> nYawRateErrorActual/1  "<nYawRateErrorActual>"
  Bus Selector10/3 -> aCamberFL/1  "<aCamberFL>"
  Bus Selector9/3 -> MTorqueVectoringRL/1  "<MTorqueVectoringRL>"
  INV2_Recieve_1/1 -> Bus Selector21/1
  Bus Selector9/6 -> MTorqueDistributionFR/1  "<MTorqueDistributionFR>"
  Bus Selector5/8 -> tIMUError/1  "<tIMUError>"
  Bus Selector/2 -> MFRFinal/1  "<MFRFinal>"
  Bus Selector11/2 -> BTVOnOW/1  "<BTVOnOW>"
  Bus Selector5/3 -> xDamperFL/1  "<xDamperFL>"
  Bus Selector14/4 -> PInvTemperatureDerateFL/1  "<PInvTemperatureDerateFL>"
  Bus Selector47/4 -> PTSTemperatureDerateRR/1  "<PTSTemperatureDerateRR>"
  Bus Selector11/1 -> BTVOnEM/1  "<BTVOnEM>"
  0x701/1 -> Bus Selector54/1
  Bus Selector8/13 -> PPCRegenRequested/1  "<PPCRegenRequested>"
  Bus Selector30/7 -> PRegenRequested/1  "<PRegenRequested>"
  Bus Selector21/6 -> CAN2 TX/7(MTorqueLimitPositiveFL)  "<MTorqueLimitPositiveFL>"
  0x210/1 -> Bus Selector5/1
  Bus Selector55/10 -> rEngineBrakingSplitOW/1  "<rEngineBrakingSplitOW>"
  Bus Selector12/7 -> PPCIntegralTermRegen/1  "<PPCIntegralTermRegen>"
  Bus Selector49/1 -> NBMSState/1  "<NBMSState>"
  Bus Selector9/1 -> MTorqueVectoringFL/1  "<MTorqueVectoringFL>"
  Bus Selector54/5 -> ESector5Remaining/1  "<ESector5Remaining>"
  0x1A2/1 -> Bus Selector18/1
  Bus Selector2/12 -> BInvErrorResetRRCAN3/1  "<BInvErrorResetRR>"
  Bus Selector12/1 -> aSteeringAngle/1  "<aSteeringAngle>"
  Bus Selector10/7 -> FTotalLateralLoadTransfer/1  "<FTotalLateralLoadTransfer>"
  Bus Selector23/1 -> CAN2 TX/9(BInvDCOnFROut)  "<BInvDCOnFROut>"
  Bus Selector7/4 -> NInvDTCFROut/1  "<NInvDTCFR>"
  Bus Selector38/4 -> NSector4Remaining/1  "<NSector4Remaining>"
  Bus Selector11/13 -> BSpinningModeOnEM/1  "<BSpinningModeOnEM>"
  Bus Selector55/3 -> PRegenMaxEM/1  "<PRegenMaxEM>"
  Bus Selector21/2 -> CAN2 TX/3(BInvEnableFL)  "<BInvEnableFL>"
  Bus Selector8/2 -> BPedalOverlap/1  "<BPedalOverlap>"
  Bus Selector5/9 -> BDataMark/1  "<BDataMark>"
  Bus Selector22/5 -> CAN1 TX/13(MTorqueLimitNegativeRR)  "<MTorqueLimitNegativeRR>"
  Bus Selector8/14 -> PDischargeLimited/1  "<PDischargeLimited>"
  Bus Selector2/10 -> BQuitInvOnFRCAN3/1  "<BQuitInvOnFR>"
  Bus Selector2/11 -> BInvErrorResetRLCAN3/1  "<BInvErrorResetRL>"
  Bus Selector/4 -> MRRFinal/1  "<MRRFinal>"
  0x223/1 -> Bus Selector8/1
  Bus Selector22/7 -> CAN1 TX/15(MInvRRFinal)  "<MRRFinal>"
  Bus Selector1/2 -> PEnergyMeter/1  "<PEnergyMeter>"
  0x216/1 -> Bus Selector15/1
  Bus Selector19/6 -> NABSMultiplierFR/1  "<NABSMultiplierFR>"
  Bus Selector20/5 -> CAN1 TX/6(MTorqueLimitNegativeRL)  "<MTorqueLimitNegativeRL>"
  0x251/1 -> Bus Selector42/1
  Bus Selector13/4 -> BErrorReset/1  "<BErrorReset>"
  Bus Selector20/2 -> CAN1 TX/3(BInvEnableRL)  "<BInvEnableRL>"
  Bus Selector21/7 -> CAN2 TX/8(MInvFLFinal)  "<MFLFinal>"
  0x703/1 -> Bus Selector38/1
  Bus Selector12/2 -> PLowCellVoltageDischargeDerate/1  "<PLowCellVoltageDischargeDerate>"
  Bus Selector11/8 -> BTCOnOW/1  "<BTCOnOW>"
  Bus Selector13/2 -> BInverterErrorRear/1  "<BInverterErrorRear>"
  Bus Selector8/16 -> BEMSDriverSignal2/1  "<BEMSDriverSignal2>"
  Bus Selector6/6 -> aSlipAngleRR/1  "<aSlipAngleRR>"
  0x205/1 -> Bus Selector2/1
  Bus Selector30/6 -> PRegenDerate/1  "<PRegenDerate>"
  Bus Selector12/5 -> MDriverRegenRequested/1  "<MDriverRegenRequested>"
  Bus Selector11/25 -> rTorqueSplit/1  "<rTorqueSplit>"
  Bus Selector31/7 -> BInvLVOn/1  "<BInvLVOn>"
  Bus Selector24/1 -> tBrakeError/1  "<tBrakeError>"
  Bus Selector54/7 -> ESector7Remaining/1  "<ESector7Remaining>"
  Bus Selector8/7 -> BxDamperRLOk/1  "<BxDamperRLOk>"
  Bus Creator/1 -> Model/2
  Bus Selector42/2 -> PMotorTemperatureDerate/1  "<PMotorTemperatureDerate>"
  Bus Selector11/14 -> BSpinningModeOnOW/1  "<BSpinningModeOnOW>"
  Bus Selector18/11 -> MRegenMax/1  "<MRegenMax>"
  From13/1 -> Bus Creator/3  "IMU"
  Bus Selector7/3 -> NInvDTCFLOut/1  "<NInvDTCFL>"
  Bus Selector19/2 -> MTorqueDistributionRR/1  "<MTorqueDistributionRR>"
  Bus Selector49/3 -> TInvFLOut/1  "<TInvFL>"
  Bus Selector13/5 -> TInvRLOut/1  "<TInvRL>"
  Bus Selector11/19 -> BBMSP0A10Out/1  "<BBMSP0A10>"
  Bus Selector19/1 -> tThrottleError/1  "<tThrottleError>"
  Bus Selector34/2 -> ESector1Remaining/1  "<ESector1Remaining>"
  Bus Selector10/5 -> aCamberRL/1  "<aCamberRL>"
  From8/1 -> CAN1_2Bus/2  "InverterFR"
  Bus Selector47/3 -> PTSTemperatureDerateFL/1  "<PTSTemperatureDerateFL>"
  0x203/1 -> Bus Selector1/1
  Bus Selector6/2 -> FTyreVerticalRR/1  "<FTyreVerticalRR>"
  Bus Selector11/27 -> NThrottleMapEM/1  "<NThrottleMapEM>"
  Bus Selector12/6 -> PPCIntegralTermDischarge/1  "<PPCIntegralTermDischarge>"
  Bus Selector18/8 -> EOffset/1  "<EOffset>"
  From11/1 -> Bus Creator/2  "DDU7"
  Bus Selector23/5 -> CAN2 TX/13(MTorqueLimitNegativeFR)  "<MTorqueLimitNegativeFR>"
  0x222/1 -> Bus Selector10/1
  Bus Selector14/6 -> IBMSHallEffectOut/1  "<IBMSHallEffect>"
  Bus Selector23/3 -> CAN2 TX/11(BInvErrorResetFR)  "<BInvErrorResetFR>"
  Bus Selector8/5 -> BxDamperFLOk/1  "<BxDamperFLOk>"
  Bus Selector3/1 -> vWheelRL/1  "<vWheelRL>"
  0x215/1 -> Bus Selector24/1
  Bus Selector19/4 -> NTractionControlMultiplierRR/1  "<NTractionControlMultiplierRR>"
  Bus Selector13/7 -> VDCAccumulatorOut/1  "<VDCAccumulator>"
  Bus Selector13/1 -> NInvState/1  "<NInvState>"
  Bus Selector42/1 -> PInvTemperatureDerateRL/1  "<PInvTemperatureDerateRL>"
  Bus Selector2/9 -> BQuitInvOnRRCAN3/1  "<BQuitInvOnRR>"
  Bus Selector55/2 -> PRegenMax/1  "<PRegenMax>"
  Bus Selector30/1 -> rSpeedRegenDerateRL/1  "<rSpeedRegenDerateRL>"
  Bus Selector10/6 -> aCamberRR/1  "<aCamberRR>"
  Bus Selector10/2 -> rSlipRatioOptimal/1  "<rSlipRatioOptimal>"
  Bus Selector22/6 -> CAN1 TX/14(MTorqueLimitPositiveRR)  "<MTorqueLimitPositiveRR>"
  0x603/1 -> Bus Selector31/1
  INV4_Recieve_1/1 -> Bus Selector23/1
  Bus Selector11/16 -> BBalancingOnOut/1  "<BBalancingOn>"
  Bus Selector3/6 -> BPageDown/1  "<BPageDown>"
  Bus Selector/6 -> PActual/1  "<PActual>"
  Bus Selector4/3 -> MPCDischargeRequested/1  "<MPCDischargeRequested>"
  Bus Selector30/8 -> PDischargeLimit/1  "<PDischargeLimit>"
  Bus Selector19/3 -> NTractionControlMultiplierRL/1  "<NTractionControlMultiplierRL>"
  Bus Selector11/23 -> NLap/1  "<NLap>"
  0x221/1 -> Bus Selector30/1
  Bus Selector3/5 -> rThrottlePedal/1  "<rThrottlePedal>"
  Bus Selector48/1 -> ESector/1  "<ESector>"
  Bus Selector14/3 -> PInvTemperatureDerateFR/1  "<PInvTemperatureDerateFR>"
  Bus Selector/5 -> IIVTSOut/1  "<IIVTS>"
  Bus Selector42/3 -> PMotorTemperatureDerateFR/1  "<PMotorTemperatureDerateFR>"
  Bus Selector42/4 -> PMotorTemperatureDerateFL/1  "<PMotorTemperatureDerateFL>"
  Bus Selector55/9 -> rEngineBrakingSplitEM/1  "<rEngineBrakingSplitEM>"
  Bus Selector/8 -> BThrottleError/1  "<BThrottleError>"
  Bus Selector11/4 -> BDrivetrainCoolingOnEM/1  "<BDrivetrainCoolingOnEM>"
  Bus Selector23/2 -> CAN2 TX/10(BInvEnableFR)  "<BInvEnableFR>"
  Bus Selector7/1 -> NInvDTCRLOut/1  "<NInvDTCRL>"
  Bus Selector55/1 -> rTorqueSplitOW/1  "<rTorqueSplitOW>"
  From7/1 -> CAN1_2Bus/1  "InverterFL"
  Bus Selector31/5 -> BMotorRBHFanOn/1  "<BMotorRBHFanOn>"
  From10/1 -> CAN1_2Bus/3  "InverterRL"
  0x252/1 -> Bus Selector35/1
  Bus Selector21/5 -> CAN2 TX/6(MTorqueLimitNegativeFL)  "<MTorqueLimitNegativeFL>"
  Bus Selector38/8 -> NSector8Remaining/1  "<NSector8Remaining>"
  Bus Selector53/1 -> ESector9Remaining/1  "<ESector9Remaining>"
  Bus Selector35/7 -> aRollAngle/1  "<aRollAngle>"
  Bus Selector18/6 -> PEngineBrakingOW/1  "<PEngineBrakingOW>"
  Bus Selector53/4 -> ESector12Remaining/1  "<ESector12Remaining>"
  Bus Selector34/3 -> ESector2Remaining/1  "<ESector2Remaining>"
  Bus Selector8/4 -> BRegenOn/1  "<BRegenOn>"
  Bus Selector31/6 -> BInverterFanOn/1  "<BInverterFanOn>"
  Bus Selector/9 -> BOverpower/1  "<BOverpower>"
  Bus Selector22/2 -> CAN1 TX/10(BInvEnableRR)  "<BInvEnableRR>"
  Bus Selector11/17 -> BBMSP0A0COut/1  "<BBMSP0A0C>"
  Bus Selector8/9 -> BIMUError/1  "<BIMUError>"
  Bus Selector8/15 -> BEMSDriverSignal1/1  "<BEMSDriverSignal1>"
  Bus Selector53/6 -> NSector2Remaining/1  "<NSector2Remaining>"
  Bus Selector2/2 -> vWheelFR/1  "<vWheelFR>"
  Bus Selector18/5 -> PEngineBrakingEM/1  "<PEngineBrakingEM>"
  Bus Selector15/5 -> rSlipRatioFRActual/1  "<rSlipRatioFRActual>"
  Bus Selector31/2 -> BBrakeLight/1  "<BBrakeLight>"
  Bus Selector55/5 -> rTVMultiplier/1  "<rTVMultiplier>"
  Bus Selector15/7 -> FTyreVerticalFR/1  "<FTyreVerticalFR>"
  Bus Selector2/8 -> BQuitInvOnFLCAN3/1  "<BQuitInvOnFL>"
  Bus Selector31/4 -> BAccuFanOn/1  "<BAccuFanOn>"
  Bus Selector13/9 -> BTVOK/1  "<BTVOK>"
  Bus Selector8/11 -> PSOCRegenDerate/1  "<PSOCRegenDerate>"
  Bus Selector48/3 -> xHeaveTravelR/1  "<xHeaveTravelR>"
  Bus Selector33/6 -> TMotorFLOut/1  "<TMotorFL>"
  Bus Selector21/3 -> CAN2 TX/4(BInvErrorResetFL)  "<BInvErrorResetFL>"
  Bus Selector30/3 -> rSpeedRegenDerateFL/1  "<rSpeedRegenDerateFL>"
  Bus Selector18/1 -> PDischargeMax/1  "<PDischargeMax>"
  Bus Selector47/1 -> PMotorTemperatureDerateRL/1  "<PMotorTemperatureDerateRL>"
  Bus Selector23/7 -> CAN2 TX/15(MInvFRFinal)  "<MFRFinal>"
  0x212/1 -> Bus Selector9/1
  Bus Selector29/5 -> VCellMaxOut/1  "<VCellMax>"
  Bus Selector11/3 -> BDrivetrainCoolingOn/1  "<BDrivetrainCoolingOn>"
  Bus Selector24/7 -> rSlipRatioRRActual/1  "<rSlipRatioRRActual>"
  Bus Selector/10 -> BDischargeAllowed/1  "<BDischargeAllowed>"
  Bus Selector11/6 -> BTCOn/1  "<BTCOn>"
  Bus Selector6/5 -> aSlipAngleRL/1  "<aSlipAngleRL>"
  Bus Selector55/13 -> BTVOn/1  "<BTVOn>"
  Bus Selector11/10 -> BEMSOnEM/1  "<BEMSOnEM>"
  Bus Selector11/24 -> NEventMode/1  "<NEventMode>"
  From12/1 -> Bus Creator/1  "STW"
  Bus Selector8/3 -> BAppsOK/1  "<BAppsOK>"
  Bus Selector24/5 -> MTractionControlFRTotal/1  "<MTractionControlFRTotal>"
  Bus Selector42/7 -> aCamberGainSteerFR/1  "<aCamberGainSteerFR>"
  Bus Selector23/4 -> CAN2 TX/12(BInvOnFROut)  "<BInvOnFROut>"
  Bus Selector8/1 -> BBrakeOn/1  "<BBrakeOn>"
  Bus Selector19/8 -> FTyreVerticalFL/1  "<FTyreVerticalFL>"
  Bus Selector2/1 -> vWheelFL/1  "<vWheelFL>"
  Bus Selector49/6 -> TCellMinOut/1  "<TCellMin>"
  Bus Selector11/21 -> BBMSP0AC0Out/1  "<BBMSP0AC0>"
  0x211/1 -> Bus Selector12/1
  Bus Selector38/7 -> NSector7Remaining/1  "<NSector7Remaining>"
  0x301/1 -> Bus Selector49/1
  Bus Selector33/5 -> TMotorRROut/1  "<TMotorRR>"
  Bus Selector34/1 -> ETotalRequested/1  "<ETotalRequested>"
  Bus Selector20/7 -> CAN1 TX/8(MInvRLFinal)  "<MRLFinal>"
  Bus Selector18/4 -> PEngineBraking/1  "<PEngineBraking>"
  Bus Selector38/9 -> ESector8Remaining/1  "<ESector8Remaining>"
  Bus Selector2/14 -> BInvErrorResetFRCAN3/1  "<BInvErrorResetFR>"
  Bus Selector49/4 -> TInvFROut/1  "<TInvFR>"
  Bus Selector49/7 -> rSplitRear/1  "<rSplitRear>"
  Bus Selector11/15 -> rSOE/1  "<rSOE>"
  Bus Selector21/1 -> CAN2 TX/2(BInvDCOnFLOut)  "<BInvDCOnFLOut>"
  Bus Selector31/1 -> BPCComplete/1  "<BPCComplete>"
  Bus Selector11/18 -> BBMSP0A0EOut/1  "<BBMSP0A0E>"
  Bus Selector18/3 -> PDischargeMaxOW/1  "<PDischargeMaxOW>"
  Bus Selector33/2 -> TInvMax/1  "<TInvMax>"
  Bus Selector54/6 -> ESector6Remaining/1  "<ESector6Remaining>"
  Bus Selector6/4 -> aSlipAngleFR/1  "<aSlipAngleFR>"
  Bus Selector4/2 -> PPCProportionalTermDischarge/1  "<PPCProportionalTermDischarge>"
  0x202/1 -> Bus Selector/1
  Bus Selector22/3 -> CAN1 TX/11(BInvErrorResetRR)  "<BInvErrorResetRR>"
  Bus Selector15/2 -> MTractionControlRRTotal/1  "<MTractionControlRRTotal>"
  Bus Selector/1 -> MFLFinal/1  "<MFLFinal>"
  0x700/1 -> Bus Selector34/1
  Bus Selector9/4 -> MTorqueVectoringRR/1  "<MTorqueVectoringRR>"
  Bus Selector5/4 -> xDamperFR/1  "<xDamperFR>"
  Bus Selector42/5 -> PMotorTemperatureDerateRR/1  "<PMotorTemperatureDerateRR>"
  Bus Selector35/4 -> aCamberGainRollR/1  "<aCamberGainRollR>"
  Bus Selector23/6 -> CAN2 TX/14(MTorqueLimitPositiveFR)  "<MTorqueLimitPositiveFR>"
  Bus Selector11/7 -> BTCOnEM/1  "<BTCOnEM>"
  Bus Selector30/5 -> PDischargeDerate/1  "<PDischargeDerate>"
  0x702/1 -> Bus Selector53/1
  Bus Selector2/5 -> rThrottlePedal1/1  "<rThrottlePedal1>"
  Bus Selector22/1 -> CAN1 TX/9(BInvDCOnRROut)  "<BInvDCOnRROut>"
  Bus Selector38/2 -> NSectorLap/1  "<NSectorLap>"
  Bus Selector18/12 -> rTorqueSplitEM/1  "<rTorqueSplitEM>"
  Bus Selector20/6 -> CAN1 TX/7(MTorqueLimitPositiveRL)  "<MTorqueLimitPositiveRL>"
  Bus Selector13/10 -> sSector/1  "<sSector>"
  Model/1 -> Goto17/1
  Bus Selector9/5 -> MTorqueDistributionFL/1  "<MTorqueDistributionFL>"
  Bus Selector30/2 -> rSpeedRegenDerateFR/1  "<rSpeedRegenDerateFR>"
  Bus Selector14/1 -> sChassis/1  "<sChassis>"
  Bus Selector47/5 -> PTSTemperatureDerateRL/1  "<PTSTemperatureDerateRL>"
  Bus Selector2/7 -> BQuitInvOnRLCAN3/1  "<BQuitInvOnRL>"
  0x207/1 -> Bus Selector7/1
  0x250/1 -> Bus Selector14/1
  Bus Selector9/2 -> MTorqueVectoringFR/1  "<MTorqueVectoringFR>"
  Bus Selector15/6 -> rSlipRatioRLActual/1  "<rSlipRatioRLActual>"
  Bus Selector10/4 -> aCamberFR/1  "<aCamberFR>"
  Bus Selector11/11 -> BEMSOnOW/1  "<BEMSOnOW>"
  Bus Selector34/4 -> ESector3Remaining/1  "<ESector3Remaining>"
  Bus Selector35/3 -> aCamberGainRollF/1  "<aCamberGainRollF>"
  Bus Selector6/3 -> aSlipAngleFL/1  "<aSlipAngleFL>"
  Bus Selector4/8 -> NTractionControlMultiplierFR/1  "<NTractionControlMultiplierFR>"
  Bus Selector11/28 -> NThrottleMapOW/1  "<NThrottleMapOW>"
  Bus Selector18/10 -> NPCKpSelector/1  "<NPCKpSelector>"
  CAN2 RX/9(MMotorMeasuredFL) -> Bus Creator14/9  "MMotorMeasuredFL"
  CAN1 RX/11(TMotorRL) -> Bus Creator17/11  "TMotorRL"
  CAN1 RX/2(BInvDCOnRLIn) -> Bus Creator17/2  "BInvDCOnRLIn"
  CAN2 RX/19(BQuitInvOnFR) -> Bus Creator15/6  "BQuitInvOnFR"
  CAN1 RX/19(BQuitInvOnRR) -> Bus Creator19/6  "BQuitInvOnRR"
  CAN1 RX/4(BInvOnRLIn) -> Bus Creator17/4  "BInvOnRLIn"
  CAN2 RX/3(BInvErrorFL) -> Bus Creator14/3  "BInvErrorFL"
  CAN1 RX/18(BInvQuitDcOnRR) -> Bus Creator19/5  "BInvQuitDcOnRR"
  CAN1 RX/13(TInvRL) -> Bus Creator17/13  "TInvRL"
  CAN2 RX/24(TMotorFR) -> Bus Creator15/11  "TMotorFR"
  CAN1 RX/23(NInvDCTRR) -> Bus Creator19/10  "NInvDTCRR"
  CAN2 RX/13(TInvFL) -> Bus Creator14/13  "TInvFL"
  CAN1 RX/15(BInvDCOnRRIn) -> Bus Creator19/2  "BInvDCOnRRIn"
  CAN2 RX/26(TInvFR) -> Bus Creator15/13  "TInvFR"
  Bus Creator18/1 -> [BMS]
  CAN2 RX/11(TMotorFL) -> Bus Creator14/11  "TMotorFL"
  CAN1 RX/20(BInvSysReadyRR) -> Bus Creator19/7  "BInvSysReadyRR"
  CAN1 RX/7(BInvSysReadyRL) -> Bus Creator17/7  "BInvSysReadyRL"
  Bus Creator14/1 -> [InverterFL]
  Bus Creator15/1 -> [InverterFR]
  CAN2 RX/20(BInvSysReadyFR) -> Bus Creator15/7  "BInvSysReadyFR"
  CAN2 RX/6(BQuitInvOnFL) -> Bus Creator14/6  "BQuitInvOnFL"
  CAN2 RX/18(BInvQuitDcOnFR) -> Bus Creator15/5  "BInvQuitDcOnFR"
  CAN2 RX/5(BInvQuitDcOnFL) -> Bus Creator14/5  "BInvQuitDcOnFL"
  CAN2 RX/23(NInvDCTFR) -> Bus Creator15/10  "NInvDTCFR"
  CAN2 RX/2(BInvDCOnFLIn) -> Bus Creator14/2  "BInvDCOnFLIn"
  CAN1 RX/14(nMotorRR) -> Bus Creator19/1  "nMotorRR"
  CAN1 RX/22(MMotorMeasuredRR) -> Bus Creator19/9  "MMotorMeasuredRR"
  CAN2 RX/12(VDCInvFL) -> Bus Creator14/12  "VDCInvFL"
  CAN1 RX/17(BInvOnRRIn) -> Bus Creator19/4  "BInvOnRRIn"
  CAN1 RX/21(BInvWarnRR) -> Bus Creator19/8  "BInvWarnRR"
  CAN2 RX/4(BInvOnFLIn) -> Bus Creator14/4  "BInvOnFLIn"
  CAN1 RX/9(MMotorMeasuredRL) -> Bus Creator17/9  "MMotorMeasuredRL"
  CAN2 RX/10(NInvDCTFL) -> Bus Creator14/10  "NInvDTCFL"
  CAN1 RX/16(BInvErrorRR) -> Bus Creator19/3  "BInvErrorRR"
  CAN1 RX/10(NInvDCTRL) -> Bus Creator17/10  "NInvDTCRL"
  CAN2 RX/1(nMotorFL) -> Bus Creator14/1  "nMotorFL"
  CAN1 RX/6(BQuitInvOnRL) -> Bus Creator17/6  "BQuitInvOnRL"
  Bus Creator17/1 -> [InverterRL]
  CAN2 RX/22(MMotorMeasuredFR) -> Bus Creator15/9  "MMotorMeasuredFR"
  CAN1 RX/8(BInvWarnRL) -> Bus Creator17/8  "BInvWarnRL"
  CAN2 RX/25(VDCInvFR) -> Bus Creator15/12  "VDCInvFR"
  CAN2 RX/14(nMotorFR) -> Bus Creator15/1  "nMotorFR"
  CAN1 RX/24(TMotorRR) -> Bus Creator19/11  "TMotorRR"
  CAN2 RX/15(BInvDCOnFRIn) -> Bus Creator15/2  "BInvDCOnFRIn"
  CAN1 RX/26(TInvRR) -> Bus Creator19/13  "TInvRR"
  CAN2 RX/21(BInvWarnFR) -> Bus Creator15/8  "BInvWarnFR"
  CAN2 RX/8(BInvWarnFL) -> Bus Creator14/8  "BInvWarnFL"
  CAN2 RX/16(BInvErrorFR) -> Bus Creator15/3  "BInvErrorFR"
  CAN2 RX/7(BInvSysReadyFL) -> Bus Creator14/7  "BInvSysReadyFL"
  CAN1 RX/1(nMotorRL) -> Bus Creator17/1  "nMotorRL"
  CAN1 RX/25(VDCInvRR) -> Bus Creator19/12  "VDCInvRR"
  CAN1 RX/3(BInvErrorRL) -> Bus Creator17/3  "BInvErrorRL"
  CAN2 RX/17(BInvOnFRIn) -> Bus Creator15/4  "BInvOnFRIn"
  Bus Creator19/1 -> [InverterRR]
  CAN1 RX/12(VDCInvRL) -> Bus Creator17/12  "VDCInvRL"
  CAN1 RX/5(BInvQuitDcOnRL) -> Bus Creator17/5  "BInvQuitDcOnRL"
  Bus Creator5/1 -> [IMU]
  Bus Creator1/1 -> [DDU7]
  Bus Creator6/1 -> [STW]
  CAN3 RX/17(BSteeringWheelButton1) -> Bus Creator6/1
  CAN3 RX/18(BSteeringWheelButton2) -> Bus Creator6/2
  CAN3 RX/19(BSteeringWheelButton3) -> Bus Creator6/3
  CAN3 RX/20(BSteeringWheelButton4) -> Bus Creator6/4
  CAN3 RX/21(NPageSelectRotary) -> Bus Creator6/5
  CAN3 RX/22(NParameterRotary) -> Bus Creator6/6
  CAN3 RX/23(NEventModeRotary) -> Bus Creator6/7
  CAN3 RX/24(VRegenPaddle1) -> Bus Creator6/8
  CAN3 RX/13(nYawRateIMU) -> Bus Creator5/6
  CAN3 RX/12(gLongitudingalIMU) -> Bus Creator5/5
  CAN3 RX/11(gLateralIMU) -> Bus Creator5/4
  CAN3 RX/10(vLongitudinalIMU) -> Bus Creator5/3
  CAN3 RX/9(gVerticalIMU) -> Bus Creator5/2
  CAN3 RX/8(vLateralIMU) -> Bus Creator5/1
  CAN3 RX/14(gSlipIMU) -> Terminator5/1
  CAN3 RX/15(nPitchIMU) -> Terminator4/1
  CAN3 RX/16(nRollIMU) -> Terminator3/1
  CAN3 RX/7(VDamperPotentiometerFL) -> Bus Creator1/8
  CAN3 RX/6(VDamperPotentiometerFR) -> Bus Creator1/7
  CAN3 RX/5(VBrakeR) -> Bus Creator1/6
  CAN3 RX/4(VBrakeF) -> Bus Creator1/5
  CAN3 RX/3(VThrottlePedal2) -> Bus Creator1/4
  CAN3 RX/2(VThrottlePedal1) -> Bus Creator1/3
  CAN3 RX/1(VSteeringAngle) -> Bus Creator1/2
  Constant1/1 -> Bus Creator1/1
  CAN3 RX/26(ID) -> Data Type Conversion/1
  CAN3 RX/27(Length) -> Data Type Conversion1/1
  CAN3 RX/25(VRegenPaddle2) -> Bus Creator6/9
  Data Type Conversion/1 -> [RXIDCAN3]
  Data Type Conversion1/1 -> [RXDLCAN3]
  CAN4 RX/18(ID) -> Data Type Conversion2/1
  Data Type Conversion3/1 -> [RXDLCAN4]
  Data Type Conversion2/1 -> [RXIDCAN4]
  CAN4 RX/19(Length) -> Data Type Conversion3/1
  CAN4 RX/1(IIVTS) -> Bus Creator18/1
  CAN4 RX/2(IBMSHallEffect) -> Bus Creator18/2
  CAN4 RX/3(VDCAccumulator) -> Bus Creator18/3
  CAN4 RX/4(TCellMin) -> Bus Creator18/4
  CAN4 RX/5(VCellAverage) -> Bus Creator18/5
  CAN4 RX/6(VCellMax) -> Bus Creator18/6
  CAN4 RX/7(TCellMax) -> Bus Creator18/7
  CAN4 RX/8(IBMSDCL) -> Bus Creator18/8
  CAN4 RX/9(VCellMin) -> Bus Creator18/9
  CAN4 RX/10(RCellAverage) -> Bus Creator18/10
  CAN4 RX/11(BBalancingOn) -> Bus Creator18/11
  CAN4 RX/12(BBMSP0A0C) -> Bus Creator18/12
  CAN4 RX/13(BBMSP0A0E) -> Bus Creator18/13
  CAN4 RX/14(BBMSP0A10) -> Bus Creator18/14
  CAN4 RX/15(BBMSP0A080) -> Bus Creator18/15
  CAN4 RX/16(BBMSP0A0C0) -> Bus Creator18/16
  CAN4 RX/17(BBMSP0AFA) -> Bus Creator18/17
  NOT4/1 -> CAN3 RX/Enable
  NOT1/1 -> CAN4 RX/Enable, Digital Port Write1/1
  Digital Port Read2/1 -> NOT1/1
  NOT2/1 -> CAN2 RX/Enable
  Digital Port Read3/1 -> NOT2/1
  NOT3/1 -> CAN1 RX/Enable
  Digital Port Read4/1 -> NOT3/1
  CAN2 RX/27(ID) -> Data Type Conversion4/1
  Data Type Conversion5/1 -> [RXDLCAN2]
  Data Type Conversion4/1 -> [RXIDCAN2]
  CAN2 RX/28(Length) -> Data Type Conversion5/1
  CAN1 RX/27(ID) -> Data Type Conversion6/1
  Data Type Conversion7/1 -> [RXDLCAN1]
  Data Type Conversion6/1 -> [RXIDCAN1]
  CAN1 RX/28(Length) -> Data Type Conversion7/1
  Initialize CAN1/1(MCPInitialized) -> Goto10/1
  Initialize CAN2/1(MCPInitialized) -> Goto11/1
  Initialize CAN4/1(MCPInitialized) -> Goto21/1
  From18/1 -> ?
  From19/1 -> ?
  Demux/7 -> Gain/1
  Demux/3 -> CAN Tx2/8(VADC3)
  Demux/1 -> CAN Tx2/6(VADC1)
  [VRRGearboxPressureSensor] -> CAN Tx2/4(VRRGearboxPressureSensor)
  [VRLGearboxPressureSensor] -> CAN Tx2/5(VRLGearboxPressureSensor)
  Gain/1 -> CAN Tx2/12(VADC7)
  Demux/2 -> CAN Tx2/7(VADC2)
  Demux/6 -> CAN Tx2/11(VADC6)
  [CAN3Initialized] -> CAN Tx2/1(MCPInitialized)
  [VFRGearboxPressureSensor] -> CAN Tx2/2(VFRGearboxPressureSensor)
  Demux/4 -> CAN Tx2/9(VADC4)
  [VFLGearboxPressureSensor] -> CAN Tx2/3(VFLGearboxPressureSensor)
  [VADCs3V3] -> Demux/1
  Demux/5 -> CAN Tx2/10(VADC5)
  [RXIDCAN2] -> CAN Tx2/14(Number2)
  [RXIDCAN3] -> CAN Tx2/15(Number3)
  [RXIDCAN4] -> CAN Tx2/16(Number4)
  [RXIDCAN1] -> CAN Tx2/13(Number1)
  [RXIDCAN4] -> CAN Tx3/16(Number4)
  [RXIDCAN2] -> CAN Tx3/14(Number2)
  [CAN4Initialized] -> ?
  [RXIDCAN3] -> CAN Tx3/15(Number3)
  [RXIDCAN1] -> CAN Tx3/13(Number1)
  Initialize CAN5/1(MCPInitialized) -> [CAN4Initialized]
  Constant/1 -> Unit Delay5/1
  Unit Delay5/1 -> Unit Delay1/1
  Unit Delay1/1 -> CAN Tx3/1(MCPInitialized)
